simulink model "DYN_6DOF"  (R2018b)
(part 7 of 18)

+ 2*IPy6*the3_dot*cos(the2)*cos(the5)*sin(the3)*sin(the5)*sin(the6) + 2*IPy6*the3_dot*cos(the3)*cos(the5)*sin(the2)*sin(the5)*sin(the6) + IPy6*the5_dot*cos(the2)*cos(the6)*sin(the3)*sin(the4)*sin(the5) + IPy6*the5_dot*cos(the3)*cos(the6)*sin(the2)*sin(the4)*sin(the5) + IPy6*the6_dot*cos(the2)*cos(the5)*sin(the3)*sin(the4)*sin(the6) + IPy6*the6_dot*cos(the3)*cos(the5)*sin(the2)*sin(the4)*sin(the6) + 2*IPy6*the6_dot*cos(the5)*cos(the6)*sin(the2)*sin(the3)*sin(the5) + Ixx5*the2_dot*cos(the4)*cos(the5)*sin(the2)*sin(the3)*sin(the5) + Ixx5*the3_dot*cos(the4)*cos(the5)*sin(the2)*sin(the3)*sin(the5) + Ixx5*the4_dot*cos(the2)*cos(the5)*sin(the3)*sin(the4)*sin(the5) + Ixx5*the4_dot*cos(the3)*cos(the5)*sin(the2)*sin(the4)*sin(the5) - Iyy5*the2_dot*cos(the4)*cos(the5)*sin(the2)*sin(the3)*sin(the5) - Iyy5*the3_dot*cos(the4)*cos(the5)*sin(the2)*sin(the3)*sin(the5) + Iyy6*the2_dot*cos(the4)*cos(the5)*sin(the2)*sin(the3)*sin(the5) - Iyy5*the4_dot*cos(the2)*cos(the5)*sin(the3)*sin(the4)*sin(the5) - Iyy5*the4_dot*cos(the3)*cos(the5)*sin(the2)*sin(the4)*sin(the5) + Iyy6*the3_dot*cos(the4)*cos(the5)*sin(the2)*sin(the3)*sin(the5) + Iyy6*the4_dot*cos(the2)*cos(the5)*sin(the3)*sin(the4)*sin(the5) + Iyy6*the4_dot*cos(the3)*cos(the5)*sin(the2)*sin(the4)*sin(the5) - Izz6*the2_dot*cos(the4)*cos(the5)*sin(the2)*sin(the3)*sin(the5) - Izz6*the3_dot*cos(the4)*cos(the5)*sin(the2)*sin(the3)*sin(the5) - Izz6*the4_dot*cos(the2)*cos(the5)*sin(the3)*sin(the4)*sin(the5) - Izz6*the4_dot*cos(the3)*cos(the5)*sin(the2)*sin(the4)*sin(the5) + 2*m5*the5_dot*x5^2*cos(the2)*cos(the3)*cos(the5)*sin(the5) - 2*m6*the6_dot*x6^2*cos(the2)*cos(the3)*cos(the6)*sin(the6) - 2*m5*the5_dot*y5^2*cos(the2)*cos(the3)*cos(the5)*sin(the5) + 2*m6*the5_dot*y6^2*cos(the2)*cos(the3)*cos(the5)*sin(the5) + 2*m6*the6_dot*y6^2*cos(the2)*cos(the3)*cos(the6)*sin(the6) - 2*m6*the5_dot*z6^2*cos(the2)*cos(the3)*cos(the5)*sin(the5) + IPz6*the2_dot*cos(the5)*sin(the2)*sin(the3)*sin(the4)*sin(the6) + IPz6*the3_dot*cos(the5)*sin(the2)*sin(the3)*sin(the4)*sin(the6) + IPz6*the5_dot*cos(the2)*sin(the3)*sin(the4)*sin(the5)*sin(the6) + IPz6*the5_dot*cos(the3)*sin(the2)*sin(the4)*sin(the5)*sin(the6) + 2*IPz6*the6_dot*cos(the5)*sin(the2)*sin(the3)*sin(the5)*sin(the6) + a3*m4*the4_dot*y4*cos(the2)*cos(the3)*cos(the4) + a2*m5*the5_dot*y5*cos(the2)*cos(the4)*cos(the5) + a2*m6*the4_dot*y6*cos(the2)*cos(the4)*cos(the6) + a1*m6*the6_dot*y6*cos(the4)*cos(the5)*cos(the6) - a3*m5*the4_dot*z5*cos(the2)*cos(the3)*cos(the4) + a2*m6*the5_dot*z6*cos(the2)*cos(the4)*cos(the5) + d4*m4*the2_dot*x4*cos(the2)*cos(the3)*cos(the4) + d4*m4*the3_dot*x4*cos(the2)*cos(the3)*cos(the4) - 2*m5*the5_dot*x5^2*cos(the5)*sin(the2)*sin(the3)*sin(the5) + m6*the6_dot*x6^2*cos(the2)*sin(the3)*sin(the4)*sin(the5) + m6*the6_dot*x6^2*cos(the3)*sin(the2)*sin(the4)*sin(the5) + 2*m6*the6_dot*x6^2*cos(the6)*sin(the2)*sin(the3)*sin(the6) + 2*m5*the5_dot*y5^2*cos(the5)*sin(the2)*sin(the3)*sin(the5) - 2*m6*the5_dot*y6^2*cos(the5)*sin(the2)*sin(the3)*sin(the5) - m6*the6_dot*y6^2*cos(the2)*sin(the3)*sin(the4)*sin(the5) - m6*the6_dot*y6^2*cos(the3)*sin(the2)*sin(the4)*sin(the5) - 2*m6*the6_dot*y6^2*cos(the6)*sin(the2)*sin(the3)*sin(the6) + 2*m6*the5_dot*z6^2*cos(the5)*sin(the2)*sin(the3)*sin(the5) + a3*m4*the2_dot*x4*cos(the2)*cos(the4)*sin(the3) + a3*m4*the2_dot*x4*cos(the3)*cos(the4)*sin(the2) + a3*m4*the3_dot*x4*cos(the2)*cos(the4)*sin(the3) + a3*m4*the3_dot*x4*cos(the3)*cos(the4)*sin(the2) + a3*m4*the4_dot*x4*cos(the2)*cos(the3)*sin(the4) + a2*m5*the2_dot*x5*cos(the4)*cos(the5)*sin(the2) + a2*m5*the4_dot*x5*cos(the2)*cos(the5)*sin(the4) + a2*m5*the5_dot*x5*cos(the2)*cos(the4)*sin(the5) + a2*m6*the4_dot*x6*cos(the2)*cos(the4)*sin(the6) + a1*m6*the4_dot*x6*cos(the5)*cos(the6)*sin(the4) + a2*m6*the6_dot*x6*cos(the2)*cos(the6)*sin(the4) + a1*m6*the5_dot*x6*cos(the4)*cos(the6)*sin(the5) + a1*m6*the6_dot*x6*cos(the4)*cos(the5)*sin(the6) + 2*IPz6*the2_dot*cos(the2)*cos(the3)*cos(the4)*cos(the5)^2*cos(the6) + 2*IPz6*the3_dot*cos(the2)*cos(the3)*cos(the4)*cos(the5)^2*cos(the6) - d4*m4*the2_dot*y4*cos(the2)*cos(the3)*sin(the4) - d4*m4*the3_dot*y4*cos(the2)*cos(the3)*sin(the4) - d4*m4*the4_dot*y4*cos(the2)*cos(the4)*sin(the3) - d4*m4*the4_dot*y4*cos(the3)*cos(the4)*sin(the2) + d4*m5*the2_dot*z5*cos(the2)*cos(the3)*sin(the4) + d4*m5*the3_dot*z5*cos(the2)*cos(the3)*sin(the4) + d4*m5*the4_dot*z5*cos(the2)*cos(the4)*sin(the3) + d4*m5*the4_dot*z5*cos(the3)*cos(the4)*sin(the2) - m5*the2_dot*x5*y5*cos(the2)*cos(the3)*cos(the4) - m5*the3_dot*x5*y5*cos(the2)*cos(the3)*cos(the4) + m4*the2_dot*x4*z4*cos(the2)*cos(the3)*cos(the4) + m4*the3_dot*x4*z4*cos(the2)*cos(the3)*cos(the4) - 2*m6*the5_dot*x6*z6*cos(the2)*cos(the3)*cos(the6) - a3*m4*the2_dot*y4*cos(the2)*sin(the3)*sin(the4) - a3*m4*the2_dot*y4*cos(the3)*sin(the2)*sin(the4) - a3*m4*the3_dot*y4*cos(the2)*sin(the3)*sin(the4) - a3*m4*the3_dot*y4*cos(the3)*sin(the2)*sin(the4) - a3*m4*the4_dot*y4*cos(the4)*sin(the2)*sin(the3) - a2*m5*the2_dot*y5*cos(the4)*sin(the2)*sin(the5) - a2*m5*the4_dot*y5*cos(the2)*sin(the4)*sin(the5) - a2*m6*the2_dot*y6*cos(the6)*sin(the2)*sin(the4) - a1*m6*the4_dot*y6*cos(the5)*sin(the4)*sin(the6) - a2*m6*the6_dot*y6*cos(the2)*sin(the4)*sin(the6) - a1*m6*the5_dot*y6*cos(the4)*sin(the5)*sin(the6) + a3*m5*the2_dot*z5*cos(the2)*sin(the3)*sin(the4) + a3*m5*the2_dot*z5*cos(the3)*sin(the2)*sin(the4) + a3*m5*the3_dot*z5*cos(the2)*sin(the3)*sin(the4) + a3*m5*the3_dot*z5*cos(the3)*sin(the2)*sin(the4) + a3*m5*the4_dot*z5*cos(the4)*sin(the2)*sin(the3) - a2*m6*the2_dot*z6*cos(the4)*sin(the2)*sin(the5) - a2*m6*the4_dot*z6*cos(the2)*sin(the4)*sin(the5) - 2*IPy6*the2_dot*cos(the2)*cos(the3)*cos(the4)*cos(the5)^2*sin(the6) - 2*IPy6*the3_dot*cos(the2)*cos(the3)*cos(the4)*cos(the5)^2*sin(the6) - 2*IPy6*the6_dot*cos(the2)*cos(the4)*cos(the5)^2*cos(the6)*sin(the3) - 2*IPy6*the6_dot*cos(the3)*cos(the4)*cos(the5)^2*cos(the6)*sin(the2) - 2*Ixx6*the5_dot*cos(the2)*cos(the3)*cos(the5)*cos(the6)^2*sin(the5) - 2*Ixx6*the6_dot*cos(the2)*cos(the3)*cos(the5)^2*cos(the6)*sin(the6) + 2*Iyy6*the5_dot*cos(the2)*cos(the3)*cos(the5)*cos(the6)^2*sin(the5) + 2*Iyy6*the6_dot*cos(the2)*cos(the3)*cos(the5)^2*cos(the6)*sin(the6) - d4*m4*the2_dot*x4*cos(the4)*sin(the2)*sin(the3) - d4*m4*the3_dot*x4*cos(the4)*sin(the2)*sin(the3) - d4*m4*the4_dot*x4*cos(the2)*sin(the3)*sin(the4) - d4*m4*the4_dot*x4*cos(the3)*sin(the2)*sin(the4) - m4*the2_dot*y4*z4*cos(the2)*cos(the3)*sin(the4) - m4*the3_dot*y4*z4*cos(the2)*cos(the3)*sin(the4) - m4*the4_dot*y4*z4*cos(the2)*cos(the4)*sin(the3) - m4*the4_dot*y4*z4*cos(the3)*cos(the4)*sin(the2) + 2*m6*the5_dot*y6*z6*cos(the2)*cos(the3)*sin(the6) - a3*m4*the4_dot*x4*sin(the2)*sin(the3)*sin(the4) - a2*m6*the2_dot*x6*sin(the2)*sin(the4)*sin(the6) - 2*IPx6*the2_dot*cos(the2)*cos(the3)*cos(the6)^2*sin(the4)*sin(the5) - 2*IPx6*the3_dot*cos(the2)*cos(the3)*cos(the6)^2*sin(the4)*sin(the5) - 2*IPx6*the2_dot*cos(the2)*cos(the5)^2*cos(the6)*sin(the3)*sin(the6) - 2*IPx6*the2_dot*cos(the3)*cos(the5)^2*cos(the6)*sin(the2)*sin(the6) - 2*IPx6*the4_dot*cos(the2)*cos(the4)*cos(the6)^2*sin(the3)*sin(the5) - 2*IPx6*the4_dot*cos(the3)*cos(the4)*cos(the6)^2*sin(the2)*sin(the5) - 2*IPx6*the3_dot*cos(the2)*cos(the5)^2*cos(the6)*sin(the3)*sin(the6) - 2*IPx6*the3_dot*cos(the3)*cos(the5)^2*cos(the6)*sin(the2)*sin(the6) - 2*IPx6*the5_dot*cos(the2)*cos(the5)*cos(the6)^2*sin(the3)*sin(the4) - 2*IPx6*the5_dot*cos(the3)*cos(the5)*cos(the6)^2*sin(the2)*sin(the4) - 2*IPz6*the2_dot*cos(the4)*cos(the5)^2*cos(the6)*sin(the2)*sin(the3) - 2*IPz6*the3_dot*cos(the4)*cos(the5)^2*cos(the6)*sin(the2)*sin(the3) - 2*IPz6*the4_dot*cos(the2)*cos(the5)^2*cos(the6)*sin(the3)*sin(the4) - 2*IPz6*the4_dot*cos(the3)*cos(the5)^2*cos(the6)*sin(the2)*sin(the4) - 2*IPz6*the6_dot*cos(the2)*cos(the4)*cos(the5)^2*sin(the3)*sin(the6) - 2*IPz6*the6_dot*cos(the3)*cos(the4)*cos(the5)^2*sin(the2)*sin(the6) + d4*m4*the2_dot*y4*sin(the2)*sin(the3)*sin(the4) + d4*m4*the3_dot*y4*sin(the2)*sin(the3)*sin(the4) - d4*m5*the2_dot*z5*sin(the2)*sin(the3)*sin(the4) - d4*m5*the3_dot*z5*sin(the2)*sin(the3)*sin(the4) + m5*the2_dot*x5*y5*cos(the4)*sin(the2)*sin(the3) + m5*the3_dot*x5*y5*cos(the4)*sin(the2)*sin(the3) + m5*the4_dot*x5*y5*cos(the2)*sin(the3)*sin(the4) + m5*the4_dot*x5*y5*cos(the3)*sin(the2)*sin(the4) - m4*the2_dot*x4*z4*cos(the4)*sin(the2)*sin(the3) - m4*the3_dot*x4*z4*cos(the4)*sin(the2)*sin(the3) - m4*the4_dot*x4*z4*cos(the2)*sin(the3)*sin(the4) - m4*the4_dot*x4*z4*cos(the3)*sin(the2)*sin(the4) + 2*m6*the5_dot*x6*z6*cos(the6)*sin(the2)*sin(the3) + 2*IPy6*the2_dot*cos(the4)*cos(the5)^2*sin(the2)*sin(the3)*sin(the6) + 2*IPy6*the3_dot*cos(the4)*cos(the5)^2*sin(the2)*sin(the3)*sin(the6) + 2*IPy6*the4_dot*cos(the2)*cos(the5)^2*sin(the3)*sin(the4)*sin(the6) + 2*IPy6*the4_dot*cos(the3)*cos(the5)^2*sin(the2)*sin(the4)*sin(the6) + 2*Ixx6*the5_dot*cos(the5)*cos(the6)^2*sin(the2)*sin(the3)*sin(the5) + 2*Ixx6*the6_dot*cos(the2)*cos(the6)^2*sin(the3)*sin(the4)*sin(the5) + 2*Ixx6*the6_dot*cos(the3)*cos(the6)^2*sin(the2)*sin(the4)*sin(the5) + 2*Ixx6*the6_dot*cos(the5)^2*cos(the6)*sin(the2)*sin(the3)*sin(the6) - 2*Iyy6*the5_dot*cos(the5)*cos(the6)^2*sin(the2)*sin(the3)*sin(the5) - 2*Iyy6*the6_dot*cos(the2)*cos(the6)^2*sin(the3)*sin(the4)*sin(the5) - 2*Iyy6*the6_dot*cos(the3)*cos(the6)^2*sin(the2)*sin(the4)*sin(the5) - 2*Iyy6*the6_dot*cos(the5)^2*cos(the6)*sin(the2)*sin(the3)*sin(the6) + 2*m5*the5_dot*x5^2*cos(the2)*cos(the4)*cos(the5)^2*sin(the3) + 2*m5*the5_dot*x5^2*cos(the3)*cos(the4)*cos(the5)^2*sin(the2) - m6*the5_dot*x6^2*cos(the2)*cos(the4)*cos(the6)^2*sin(the3) - m6*the5_dot*x6^2*cos(the3)*cos(the4)*cos(the6)^2*sin(the2) - 2*m5*the5_dot*y5^2*cos(the2)*cos(the4)*cos(the5)^2*sin(the3) - 2*m5*the5_dot*y5^2*cos(the3)*cos(the4)*cos(the5)^2*sin(the2) + 2*m6*the5_dot*y6^2*cos(the2)*cos(the4)*cos(the5)^2*sin(the3) + 2*m6*the5_dot*y6^2*cos(the3)*cos(the4)*cos(the5)^2*sin(the2) + m6*the5_dot*y6^2*cos(the2)*cos(the4)*cos(the6)^2*sin(the3) + m6*the5_dot*y6^2*cos(the3)*cos(the4)*cos(the6)^2*sin(the2) - 2*m6*the5_dot*z6^2*cos(the2)*cos(the4)*cos(the5)^2*sin(the3) - 2*m6*the5_dot*z6^2*cos(the3)*cos(the4)*cos(the5)^2*sin(the2) + m4*the2_dot*y4*z4*sin(the2)*sin(the3)*sin(the4) + m4*the3_dot*y4*z4*sin(the2)*sin(the3)*sin(the4) - 2*m6*the5_dot*y6*z6*sin(the2)*sin(the3)*sin(the6) + 2*IPx6*the2_dot*cos(the6)^2*sin(the2)*sin(the3)*sin(the4)*sin(the5) + 2*IPx6*the3_dot*cos(the6)^2*sin(the2)*sin(the3)*sin(the4)*sin(the5) - 4*m6*the5_dot*y6*z6*cos(the2)*cos(the3)*cos(the5)^2*sin(the6) - 2*m5*the2_dot*x5*y5*cos(the4)*cos(the5)^2*sin(the2)*sin(the3) - 2*m5*the3_dot*x5*y5*cos(the4)*cos(the5)^2*sin(the2)*sin(the3) - 2*m5*the4_dot*x5*y5*cos(the2)*cos(the5)^2*sin(the3)*sin(the4) - 2*m5*the4_dot*x5*y5*cos(the3)*cos(the5)^2*sin(the2)*sin(the4) - 4*m6*the5_dot*x6*z6*cos(the5)^2*cos(the6)*sin(the2)*sin(the3) + 2*m6*the5_dot*x6^2*cos(the2)*cos(the4)*cos(the5)^2*cos(the6)^2*sin(the3) + 2*m6*the5_dot*x6^2*cos(the3)*cos(the4)*cos(the5)^2*cos(the6)^2*sin(the2) - 2*m6*the5_dot*y6^2*cos(the2)*cos(the4)*cos(the5)^2*cos(the6)^2*sin(the3) - 2*m6*the5_dot*y6^2*cos(the3)*cos(the4)*cos(the5)^2*cos(the6)^2*sin(the2) + 4*m6*the5_dot*y6*z6*cos(the5)^2*sin(the2)*sin(the3)*sin(the6) - 4*IPx6*the5_dot*cos(the2)*cos(the3)*cos(the5)*cos(the6)*sin(the5)*sin(the6) - 4*IPz6*the5_dot*cos(the2)*cos(the4)*cos(the5)*cos(the6)*sin(the3)*sin(the5) - 4*IPz6*the5_dot*cos(the3)*cos(the4)*cos(the5)*cos(the6)*sin(the2)*sin(the5) + 4*m6*the6_dot*x6*y6*cos(the2)*cos(the3)*cos(the5)^2*cos(the6)^2 + 4*IPy6*the5_dot*cos(the2)*cos(the4)*cos(the5)*sin(the3)*sin(the5)*sin(the6) + 4*IPy6*the5_dot*cos(the3)*cos(the4)*cos(the5)*sin(the2)*sin(the5)*sin(the6) + Ixx6*the2_dot*cos(the2)*cos(the3)*cos(the6)*sin(the4)*sin(the5)*sin(the6) + Ixx6*the3_dot*cos(the2)*cos(the3)*cos(the6)*sin(the4)*sin(the5)*sin(the6) + Ixx6*the4_dot*cos(the2)*cos(the4)*cos(the6)*sin(the3)*sin(the5)*sin(the6) + Ixx6*the4_dot*cos(the3)*cos(the4)*cos(the6)*sin(the2)*sin(the5)*sin(the6) + Ixx6*the5_dot*cos(the2)*cos(the5)*cos(the6)*sin(the3)*sin(the4)*sin(the6) + Ixx6*the5_dot*cos(the3)*cos(the5)*cos(the6)*sin(the2)*sin(the4)*sin(the6) - Iyy6*the2_dot*cos(the2)*cos(the3)*cos(the6)*sin(the4)*sin(the5)*sin(the6) - Iyy6*the3_dot*cos(the2)*cos(the3)*cos(the6)*sin(the4)*sin(the5)*sin(the6) - Iyy6*the4_dot*cos(the2)*cos(the4)*cos(the6)*sin(the3)*sin(the5)*sin(the6) - Iyy6*the4_dot*cos(the3)*cos(the4)*cos(the6)*sin(the2)*sin(the5)*sin(the6) - Iyy6*the5_dot*cos(the2)*cos(the5)*cos(the6)*sin(the3)*sin(the4)*sin(the6) - Iyy6*the5_dot*cos(the3)*cos(the5)*cos(the6)*sin(the2)*sin(the4)*sin(the6) + m5*the2_dot*x5^2*cos(the2)*cos(the3)*cos(the4)*cos(the5)*sin(the5) + m5*the3_dot*x5^2*cos(the2)*cos(the3)*cos(the4)*cos(the5)*sin(the5) - m5*the2_dot*y5^2*cos(the2)*cos(the3)*cos(the4)*cos(the5)*sin(the5) - m5*the3_dot*y5^2*cos(the2)*cos(the3)*cos(the4)*cos(the5)*sin(the5) + m6*the2_dot*y6^2*cos(the2)*cos(the3)*cos(the4)*cos(the5)*sin(the5) + m6*the3_dot*y6^2*cos(the2)*cos(the3)*cos(the4)*cos(the5)*sin(the5) - m6*the2_dot*z6^2*cos(the2)*cos(the3)*cos(the4)*cos(the5)*sin(the5) - m6*the3_dot*z6^2*cos(the2)*cos(the3)*cos(the4)*cos(the5)*sin(the5) + 4*IPx6*the5_dot*cos(the5)*cos(the6)*sin(the2)*sin(the3)*sin(the5)*sin(the6) + 4*IPx6*the6_dot*cos(the2)*cos(the6)*sin(the3)*sin(the4)*sin(the5)*sin(the6) + 4*IPx6*the6_dot*cos(the3)*cos(the6)*sin(the2)*sin(the4)*sin(the5)*sin(the6) - 4*m6*the6_dot*x6*y6*cos(the5)^2*cos(the6)^2*sin(the2)*sin(the3) + a3*m5*the5_dot*y5*cos(the2)*cos(the3)*cos(the4)*cos(the5) + a3*m6*the4_dot*y6*cos(the2)*cos(the3)*cos(the4)*cos(the6) + a2*m6*the6_dot*y6*cos(the2)*cos(the4)*cos(the5)*cos(the6) + a3*m6*the5_dot*z6*cos(the2)*cos(the3)*cos(the4)*cos(the5) + d4*m5*the2_dot*x5*cos(the2)*cos(the3)*cos(the4)*cos(the5) + d4*m5*the3_dot*x5*cos(the2)*cos(the3)*cos(the4)*cos(the5) - Ixx6*the2_dot*cos(the6)*sin(the2)*sin(the3)*sin(the4)*sin(the5)*sin(the6) - Ixx6*the3_dot*cos(the6)*sin(the2)*sin(the3)*sin(the4)*sin(the5)*sin(the6) + Iyy6*the2_dot*cos(the6)*sin(the2)*sin(the3)*sin(the4)*sin(the5)*sin(the6) + Iyy6*the3_dot*cos(the6)*sin(the2)*sin(the3)*sin(the4)*sin(the5)*sin(the6) - m5*the2_dot*x5^2*cos(the4)*cos(the5)*sin(the2)*sin(the3)*sin(the5) - m5*the3_dot*x5^2*cos(the4)*cos(the5)*sin(the2)*sin(the3)*sin(the5) - m5*the4_dot*x5^2*cos(the2)*cos(the5)*sin(the3)*sin(the4)*sin(the5) - m5*the4_dot*x5^2*cos(the3)*cos(the5)*sin(the2)*sin(the4)*sin(the5) + m5*the2_dot*y5^2*cos(the4)*cos(the5)*sin(the2)*sin(the3)*sin(the5) + m5*the3_dot*y5^2*cos(the4)*cos(the5)*sin(the2)*sin(the3)*sin(the5) + m5*the4_dot*y5^2*cos(the2)*cos(the5)*sin(the3)*sin(the4)*sin(the5) + m5*the4_dot*y5^2*cos(the3)*cos(the5)*sin(the2)*sin(the4)*sin(the5) - m6*the2_dot*y6^2*cos(the4)*cos(the5)*sin(the2)*sin(the3)*sin(the5) - m6*the3_dot*y6^2*cos(the4)*cos(the5)*sin(the2)*sin(the3)*sin(the5) - m6*the4_dot*y6^2*cos(the2)*cos(the5)*sin(the3)*sin(the4)*sin(the5) - m6*the4_dot*y6^2*cos(the3)*cos(the5)*sin(the2)*sin(the4)*sin(the5) + m6*the2_dot*z6^2*cos(the4)*cos(the5)*sin(the2)*sin(the3)*sin(the5) + m6*the3_dot*z6^2*cos(the4)*cos(the5)*sin(the2)*sin(the3)*sin(the5) + m6*the4_dot*z6^2*cos(the2)*cos(the5)*sin(the3)*sin(the4)*sin(the5) + m6*the4_dot*z6^2*cos(the3)*cos(the5)*sin(the2)*sin(the4)*sin(the5) + a3*m5*the2_dot*x5*cos(the2)*cos(the4)*cos(the5)*sin(the3) + a3*m5*the2_dot*x5*cos(the3)*cos(the4)*cos(the5)*sin(the2) + a3*m5*the3_dot*x5*cos(the2)*cos(the4)*cos(the5)*sin(the3) + a3*m5*the3_dot*x5*cos(the3)*cos(the4)*cos(the5)*sin(the2) + a3*m5*the4_dot*x5*cos(the2)*cos(the3)*cos(the5)*sin(the4) + a3*m5*the5_dot*x5*cos(the2)*cos(the3)*cos(the4)*sin(the5) + a2*m6*the2_dot*x6*cos(the4)*cos(the5)*cos(the6)*sin(the2) + a3*m6*the4_dot*x6*cos(the2)*cos(the3)*cos(the4)*sin(the6) + a2*m6*the4_dot*x6*cos(the2)*cos(the5)*cos(the6)*sin(the4) + a2*m6*the5_dot*x6*cos(the2)*cos(the4)*cos(the6)*sin(the5) + a3*m6*the6_dot*x6*cos(the2)*cos(the3)*cos(the6)*sin(the4) + a2*m6*the6_dot*x6*cos(the2)*cos(the4)*cos(the5)*sin(the6) - d4*m5*the2_dot*y5*cos(the2)*cos(the3)*cos(the4)*sin(the5) - d4*m5*the3_dot*y5*cos(the2)*cos(the3)*cos(the4)*sin(the5) - d4*m5*the5_dot*y5*cos(the2)*cos(the4)*cos(the5)*sin(the3) - d4*m5*the5_dot*y5*cos(the3)*cos(the4)*cos(the5)*sin(the2) - d4*m6*the2_dot*y6*cos(the2)*cos(the3)*cos(the6)*sin(the4) - d4*m6*the3_dot*y6*cos(the2)*cos(the3)*cos(the6)*sin(the4) - d4*m6*the4_dot*y6*cos(the2)*cos(the4)*cos(the6)*sin(the3) - d4*m6*the4_dot*y6*cos(the3)*cos(the4)*cos(the6)*sin(the2) - d4*m6*the2_dot*z6*cos(the2)*cos(the3)*cos(the4)*sin(the5) - d4*m6*the3_dot*z6*cos(the2)*cos(the3)*cos(the4)*sin(the5) - d4*m6*the5_dot*z6*cos(the2)*cos(the4)*cos(the5)*sin(the3) - d4*m6*the5_dot*z6*cos(the3)*cos(the4)*cos(the5)*sin(the2) - m6*the2_dot*x6*z6*cos(the2)*cos(the3)*cos(the4)*cos(the6) - m6*the3_dot*x6*z6*cos(the2)*cos(the3)*cos(the4)*cos(the6) - a3*m5*the2_dot*y5*cos(the2)*cos(the4)*sin(the3)*sin(the5) - a3*m5*the2_dot*y5*cos(the3)*cos(the4)*sin(the2)*sin(the5) - a3*m5*the3_dot*y5*cos(the2)*cos(the4)*sin(the3)*sin(the5) - a3*m5*the3_dot*y5*cos(the3)*cos(the4)*sin(the2)*sin(the5) - a3*m5*the4_dot*y5*cos(the2)*cos(the3)*sin(the4)*sin(the5) - a3*m5*the5_dot*y5*cos(the4)*cos(the5)*sin(the2)*sin(the3) - a3*m6*the2_dot*y6*cos(the2)*cos(the6)*sin(the3)*sin(the4) - a3*m6*the2_dot*y6*cos(the3)*cos(the6)*sin(the2)*sin(the4) - a2*m6*the2_dot*y6*cos(the4)*cos(the5)*sin(the2)*sin(the6) - a3*m6*the3_dot*y6*cos(the2)*cos(the6)*sin(the3)*sin(the4) - a3*m6*the3_dot*y6*cos(the3)*cos(the6)*sin(the2)*sin(the4) - a3*m6*the4_dot*y6*cos(the4)*cos(the6)*sin(the2)*sin(the3) - a2*m6*the4_dot*y6*cos(the2)*cos(the5)*sin(the4)*sin(the6) - a2*m6*the5_dot*y6*cos(the2)*cos(the4)*sin(the5)*sin(the6) - a3*m6*the6_dot*y6*cos(the2)*cos(the3)*sin(the4)*sin(the6) - a3*m6*the2_dot*z6*cos(the2)*cos(the4)*sin(the3)*sin(the5) - a3*m6*the2_dot*z6*cos(the3)*cos(the4)*sin(the2)*sin(the5) - a3*m6*the3_dot*z6*cos(the2)*cos(the4)*sin(the3)*sin(the5) - a3*m6*the3_dot*z6*cos(the3)*cos(the4)*sin(the2)*sin(the5) - a3*m6*the4_dot*z6*cos(the2)*cos(the3)*sin(the4)*sin(the5) - a3*m6*the5_dot*z6*cos(the4)*cos(the5)*sin(the2)*sin(the3) - Ixx6*the2_dot*cos(the2)*cos(the3)*cos(the4)*cos(the5)*cos(the6)^2*sin(the5) - Ixx6*the3_dot*cos(the2)*cos(the3)*cos(the4)*cos(the5)*cos(the6)^2*sin(the5) + Iyy6*the2_dot*cos(the2)*cos(the3)*cos(the4)*cos(the5)*cos(the6)^2*sin(the5) + Iyy6*the3_dot*cos(the2)*cos(the3)*cos(the4)*cos(the5)*cos(the6)^2*sin(the5) - d4*m5*the2_dot*x5*cos(the4)*cos(the5)*sin(the2)*sin(the3) - d4*m5*the3_dot*x5*cos(the4)*cos(the5)*sin(the2)*sin(the3) - d4*m5*the4_dot*x5*cos(the2)*cos(the5)*sin(the3)*sin(the4) - d4*m5*the4_dot*x5*cos(the3)*cos(the5)*sin(the2)*sin(the4) - d4*m5*the5_dot*x5*cos(the2)*cos(the4)*sin(the3)*sin(the5) - d4*m5*the5_dot*x5*cos(the3)*cos(the4)*sin(the2)*sin(the5) - d4*m6*the2_dot*x6*cos(the2)*cos(the3)*sin(the4)*sin(the6) - d4*m6*the3_dot*x6*cos(the2)*cos(the3)*sin(the4)*sin(the6) - d4*m6*the4_dot*x6*cos(the2)*cos(the4)*sin(the3)*sin(the6) - d4*m6*the4_dot*x6*cos(the3)*cos(the4)*sin(the2)*sin(the6) - d4*m6*the6_dot*x6*cos(the2)*cos(the6)*sin(the3)*sin(the4) - d4*m6*the6_dot*x6*cos(the3)*cos(the6)*sin(the2)*sin(the4) + m5*the2_dot*y5*z5*cos(the2)*cos(the3)*cos(the5)*sin(the4) + m5*the3_dot*y5*z5*cos(the2)*cos(the3)*cos(the5)*sin(the4) + m5*the4_dot*y5*z5*cos(the2)*cos(the4)*cos(the5)*sin(the3) + m5*the4_dot*y5*z5*cos(the3)*cos(the4)*cos(the5)*sin(the2) + m6*the2_dot*y6*z6*cos(the2)*cos(the3)*cos(the4)*sin(the6) + m6*the3_dot*y6*z6*cos(the2)*cos(the3)*cos(the4)*sin(the6) + m6*the6_dot*y6*z6*cos(the2)*cos(the4)*cos(the6)*sin(the3) + m6*the6_dot*y6*z6*cos(the3)*cos(the4)*cos(the6)*sin(the2) - a3*m5*the4_dot*x5*cos(the5)*sin(the2)*sin(the3)*sin(the4) - a3*m5*the5_dot*x5*cos(the4)*sin(the2)*sin(the3)*sin(the5) - a3*m6*the2_dot*x6*cos(the2)*sin(the3)*sin(the4)*sin(the6) - a3*m6*the2_dot*x6*cos(the3)*sin(the2)*sin(the4)*sin(the6) - a3*m6*the3_dot*x6*cos(the2)*sin(the3)*sin(the4)*sin(the6) - a3*m6*the3_dot*x6*cos(the3)*sin(the2)*sin(the4)*sin(the6) - a3*m6*the4_dot*x6*cos(the4)*sin(the2)*sin(the3)*sin(the6) - a3*m6*the6_dot*x6*cos(the6)*sin(the2)*sin(the3)*sin(the4) - 4*IPx6*the5_dot*cos(the2)*cos(the4)*cos(the5)^2*cos(the6)*sin(the3)*sin(the6) - 4*IPx6*the5_dot*cos(the3)*cos(the4)*cos(the5)^2*cos(the6)*sin(the2)*sin(the6) - 4*IPx6*the6_dot*cos(the2)*cos(the4)*cos(the5)*cos(the6)^2*sin(the3)*sin(the5) - 4*IPx6*the6_dot*cos(the3)*cos(the4)*cos(the5)*cos(the6)^2*sin(the2)*sin(the5) + d4*m5*the2_dot*y5*cos(the4)*sin(the2)*sin(the3)*sin(the5) + d4*m5*the3_dot*y5*cos(the4)*sin(the2)*sin(the3)*sin(the5) + d4*m5*the4_dot*y5*cos(the2)*sin(the3)*sin(the4)*sin(the5) + d4*m5*the4_dot*y5*cos(the3)*sin(the2)*sin(the4)*sin(the5) + d4*m6*the2_dot*y6*cos(the6)*sin(the2)*sin(the3)*sin(the4) + d4*m6*the3_dot*y6*cos(the6)*sin(the2)*sin(the3)*sin(the4) + d4*m6*the6_dot*y6*cos(the2)*sin(the3)*sin(the4)*sin(the6) + d4*m6*the6_dot*y6*cos(the3)*sin(the2)*sin(the4)*sin(the6) + d4*m6*the2_dot*z6*cos(the4)*sin(the2)*sin(the3)*sin(the5) + d4*m6*the3_dot*z6*cos(the4)*sin(the2)*sin(the3)*sin(the5) + d4*m6*the4_dot*z6*cos(the2)*sin(the3)*sin(the4)*sin(the5) + d4*m6*the4_dot*z6*cos(the3)*sin(the2)*sin(the4)*sin(the5) - 2*m5*the2_dot*x5*y5*cos(the2)*cos(the5)*sin(the3)*sin(the5) - 2*m5*the2_dot*x5*y5*cos(the3)*cos(the5)*sin(the2)*sin(the5) - 2*m5*the3_dot*x5*y5*cos(the2)*cos(the5)*sin(the3)*sin(the5) - 2*m5*the3_dot*x5*y5*cos(the3)*cos(the5)*sin(the2)*sin(the5) + m6*the2_dot*x6*y6*cos(the2)*cos(the3)*sin(the4)*sin(the5) + m6*the3_dot*x6*y6*cos(the2)*cos(the3)*sin(the4)*sin(the5) + m6*the4_dot*x6*y6*cos(the2)*cos(the4)*sin(the3)*sin(the5) + m6*the4_dot*x6*y6*cos(the3)*cos(the4)*sin(the2)*sin(the5) + 2*m6*the2_dot*x6*y6*cos(the2)*cos(the6)*sin(the3)*sin(the6) + 2*m6*the2_dot*x6*y6*cos(the3)*cos(the6)*sin(the2)*sin(the6) + m6*the5_dot*x6*y6*cos(the2)*cos(the5)*sin(the3)*sin(the4) + m6*the5_dot*x6*y6*cos(the3)*cos(the5)*sin(the2)*sin(the4) + 2*m6*the3_dot*x6*y6*cos(the2)*cos(the6)*sin(the3)*sin(the6) + 2*m6*the3_dot*x6*y6*cos(the3)*cos(the6)*sin(the2)*sin(the6) + m5*the2_dot*x5*z5*cos(the2)*cos(the3)*sin(the4)*sin(the5) + m5*the3_dot*x5*z5*cos(the2)*cos(the3)*sin(the4)*sin(the5) + m5*the4_dot*x5*z5*cos(the2)*cos(the4)*sin(the3)*sin(the5) + m5*the4_dot*x5*z5*cos(the3)*cos(the4)*sin(the2)*sin(the5) + m5*the5_dot*x5*z5*cos(the2)*cos(the5)*sin(the3)*sin(the4) + m5*the5_dot*x5*z5*cos(the3)*cos(the5)*sin(the2)*sin(the4) + m6*the2_dot*x6*z6*cos(the4)*cos(the6)*sin(the2)*sin(the3) + m6*the3_dot*x6*z6*cos(the4)*cos(the6)*sin(the2)*sin(the3) + m6*the4_dot*x6*z6*cos(the2)*cos(the6)*sin(the3)*sin(the4) + m6*the4_dot*x6*z6*cos(the3)*cos(the6)*sin(the2)*sin(the4) + m6*the6_dot*x6*z6*cos(the2)*cos(the4)*sin(the3)*sin(the6) + m6*the6_dot*x6*z6*cos(the3)*cos(the4)*sin(the2)*sin(the6) + a3*m5*the4_dot*y5*sin(the2)*sin(the3)*sin(the4)*sin(the5) + a3*m6*the6_dot*y6*sin(the2)*sin(the3)*sin(the4)*sin(the6) + a3*m6*the4_dot*z6*sin(the2)*sin(the3)*sin(the4)*sin(the5) + Ixx6*the2_dot*cos(the4)*cos(the5)*cos(the6)^2*sin(the2)*sin(the3)*sin(the5) + Ixx6*the3_dot*cos(the4)*cos(the5)*cos(the6)^2*sin(the2)*sin(the3)*sin(the5) + Ixx6*the4_dot*cos(the2)*cos(the5)*cos(the6)^2*sin(the3)*sin(the4)*sin(the5) + Ixx6*the4_dot*cos(the3)*cos(the5)*cos(the6)^2*sin(the2)*sin(the4)*sin(the5) - Iyy6*the2_dot*cos(the4)*cos(the5)*cos(the6)^2*sin(the2)*sin(the3)*sin(the5) - Iyy6*the3_dot*cos(the4)*cos(the5)*cos(the6)^2*sin(the2)*sin(the3)*sin(the5) - Iyy6*the4_dot*cos(the2)*cos(the5)*cos(the6)^2*sin(the3)*sin(the4)*sin(the5) - Iyy6*the4_dot*cos(the3)*cos(the5)*cos(the6)^2*sin(the2)*sin(the4)*sin(the5) + d4*m6*the2_dot*x6*sin(the2)*sin(the3)*sin(the4)*sin(the6) + d4*m6*the3_dot*x6*sin(the2)*sin(the3)*sin(the4)*sin(the6) + 2*m6*the5_dot*x6^2*cos(the2)*cos(the3)*cos(the5)*cos(the6)^2*sin(the5) + 2*m6*the6_dot*x6^2*cos(the2)*cos(the3)*cos(the5)^2*cos(the6)*sin(the6) - 2*m6*the5_dot*y6^2*cos(the2)*cos(the3)*cos(the5)*cos(the6)^2*sin(the5) - 2*m6*the6_dot*y6^2*cos(the2)*cos(the3)*cos(the5)^2*cos(the6)*sin(the6) - m5*the2_dot*y5*z5*cos(the5)*sin(the2)*sin(the3)*sin(the4) - m5*the3_dot*y5*z5*cos(the5)*sin(the2)*sin(the3)*sin(the4) - m5*the5_dot*y5*z5*cos(the2)*sin(the3)*sin(the4)*sin(the5) - m5*the5_dot*y5*z5*cos(the3)*sin(the2)*sin(the4)*sin(the5) - m6*the2_dot*y6*z6*cos(the4)*sin(the2)*sin(the3)*sin(the6) - m6*the3_dot*y6*z6*cos(the4)*sin(the2)*sin(the3)*sin(the6) - m6*the4_dot*y6*z6*cos(the2)*sin(the3)*sin(the4)*sin(the6) - m6*the4_dot*y6*z6*cos(the3)*sin(the2)*sin(the4)*sin(the6) - m6*the2_dot*x6*y6*sin(the2)*sin(the3)*sin(the4)*sin(the5) - m6*the3_dot*x6*y6*sin(the2)*sin(the3)*sin(the4)*sin(the5) - m5*the2_dot*x5*z5*sin(the2)*sin(the3)*sin(the4)*sin(the5) - m5*the3_dot*x5*z5*sin(the2)*sin(the3)*sin(the4)*sin(the5) - 2*m6*the5_dot*x6^2*cos(the5)*cos(the6)^2*sin(the2)*sin(the3)*sin(the5) - 2*m6*the6_dot*x6^2*cos(the2)*cos(the6)^2*sin(the3)*sin(the4)*sin(the5) - 2*m6*the6_dot*x6^2*cos(the3)*cos(the6)^2*sin(the2)*sin(the4)*sin(the5) - 2*m6*the6_dot*x6^2*cos(the5)^2*cos(the6)*sin(the2)*sin(the3)*sin(the6) + 2*m6*the5_dot*y6^2*cos(the5)*cos(the6)^2*sin(the2)*sin(the3)*sin(the5) + 2*m6*the6_dot*y6^2*cos(the2)*cos(the6)^2*sin(the3)*sin(the4)*sin(the5) + 2*m6*the6_dot*y6^2*cos(the3)*cos(the6)^2*sin(the2)*sin(the4)*sin(the5) + 2*m6*the6_dot*y6^2*cos(the5)^2*cos(the6)*sin(the2)*sin(the3)*sin(the6) + 2*m5*the2_dot*x5*y5*cos(the2)*cos(the3)*cos(the4)*cos(the5)^2 + 2*m5*the3_dot*x5*y5*cos(the2)*cos(the3)*cos(the4)*cos(the5)^2 + 4*m6*the5_dot*x6*z6*cos(the2)*cos(the3)*cos(the5)^2*cos(the6) + 2*m6*the2_dot*x6*y6*cos(the6)^2*sin(the2)*sin(the3)*sin(the4)*sin(the5) + 2*m6*the3_dot*x6*y6*cos(the6)^2*sin(the2)*sin(the3)*sin(the4)*sin(the5) - 2*IPx6*the2_dot*cos(the2)*cos(the3)*cos(the4)*cos(the5)*cos(the6)*sin(the5)*sin(the6) - 2*IPx6*the3_dot*cos(the2)*cos(the3)*cos(the4)*cos(the5)*cos(the6)*sin(the5)*sin(the6) + 2*Ixx6*the6_dot*cos(the2)*cos(the4)*cos(the5)*cos(the6)*sin(the3)*sin(the5)*sin(the6) + 2*Ixx6*the6_dot*cos(the3)*cos(the4)*cos(the5)*cos(the6)*sin(the2)*sin(the5)*sin(the6) - 2*Iyy6*the6_dot*cos(the2)*cos(the4)*cos(the5)*cos(the6)*sin(the3)*sin(the5)*sin(the6) - 2*Iyy6*the6_dot*cos(the3)*cos(the4)*cos(the5)*cos(the6)*sin(the2)*sin(the5)*sin(the6) + 2*IPx6*the2_dot*cos(the4)*cos(the5)*cos(the6)*sin(the2)*sin(the3)*sin(the5)*sin(the6) + 2*IPx6*the3_dot*cos(the4)*cos(the5)*cos(the6)*sin(the2)*sin(the3)*sin(the5)*sin(the6) + 2*IPx6*the4_dot*cos(the2)*cos(the5)*cos(the6)*sin(the3)*sin(the4)*sin(the5)*sin(the6) + 2*IPx6*the4_dot*cos(the3)*cos(the5)*cos(the6)*sin(the2)*sin(the4)*sin(the5)*sin(the6) + a3*m6*the6_dot*y6*cos(the2)*cos(the3)*cos(the4)*cos(the5)*cos(the6) + d4*m6*the2_dot*x6*cos(the2)*cos(the3)*cos(the4)*cos(the5)*cos(the6) + d4*m6*the3_dot*x6*cos(the2)*cos(the3)*cos(the4)*cos(the5)*cos(the6) - m6*the2_dot*x6^2*cos(the2)*cos(the3)*cos(the6)*sin(the4)*sin(the5)*sin(the6) - m6*the3_dot*x6^2*cos(the2)*cos(the3)*cos(the6)*sin(the4)*sin(the5)*sin(the6) - m6*the4_dot*x6^2*cos(the2)*cos(the4)*cos(the6)*sin(the3)*sin(the5)*sin(the6) - m6*the4_dot*x6^2*cos(the3)*cos(the4)*cos(the6)*sin(the2)*sin(the5)*sin(the6) - m6*the5_dot*x6^2*cos(the2)*cos(the5)*cos(the6)*sin(the3)*sin(the4)*sin(the6) - m6*the5_dot*x6^2*cos(the3)*cos(the5)*cos(the6)*sin(the2)*sin(the4)*sin(the6) + m6*the2_dot*y6^2*cos(the2)*cos(the3)*cos(the6)*sin(the4)*sin(the5)*sin(the6) + m6*the3_dot*y6^2*cos(the2)*cos(the3)*cos(the6)*sin(the4)*sin(the5)*sin(the6) + m6*the4_dot*y6^2*cos(the2)*cos(the4)*cos(the6)*sin(the3)*sin(the5)*sin(the6) + m6*the4_dot*y6^2*cos(the3)*cos(the4)*cos(the6)*sin(the2)*sin(the5)*sin(the6) + m6*the5_dot*y6^2*cos(the2)*cos(the5)*cos(the6)*sin(the3)*sin(the4)*sin(the6) + m6*the5_dot*y6^2*cos(the3)*cos(the5)*cos(the6)*sin(the2)*sin(the4)*sin(the6) + a3*m6*the2_dot*x6*cos(the2)*cos(the4)*cos(the5)*cos(the6)*sin(the3) + a3*m6*the2_dot*x6*cos(the3)*cos(the4)*cos(the5)*cos(the6)*sin(the2) + a3*m6*the3_dot*x6*cos(the2)*cos(the4)*cos(the5)*cos(the6)*sin(the3) + a3*m6*the3_dot*x6*cos(the3)*cos(the4)*cos(the5)*cos(the6)*sin(the2) + a3*m6*the4_dot*x6*cos(the2)*cos(the3)*cos(the5)*cos(the6)*sin(the4) + a3*m6*the5_dot*x6*cos(the2)*cos(the3)*cos(the4)*cos(the6)*sin(the5) + a3*m6*the6_dot*x6*cos(the2)*cos(the3)*cos(the4)*cos(the5)*sin(the6) - d4*m6*the2_dot*y6*cos(the2)*cos(the3)*cos(the4)*cos(the5)*sin(the6) - d4*m6*the3_dot*y6*cos(the2)*cos(the3)*cos(the4)*cos(the5)*sin(the6) - d4*m6*the6_dot*y6*cos(the2)*cos(the4)*cos(the5)*cos(the6)*sin(the3) - d4*m6*the6_dot*y6*cos(the3)*cos(the4)*cos(the5)*cos(the6)*sin(the2) - a3*m6*the2_dot*y6*cos(the2)*cos(the4)*cos(the5)*sin(the3)*sin(the6) - a3*m6*the2_dot*y6*cos(the3)*cos(the4)*cos(the5)*sin(the2)*sin(the6) - a3*m6*the3_dot*y6*cos(the2)*cos(the4)*cos(the5)*sin(the3)*sin(the6) - a3*m6*the3_dot*y6*cos(the3)*cos(the4)*cos(the5)*sin(the2)*sin(the6) - a3*m6*the4_dot*y6*cos(the2)*cos(the3)*cos(the5)*sin(the4)*sin(the6) - a3*m6*the5_dot*y6*cos(the2)*cos(the3)*cos(the4)*sin(the5)*sin(the6) - a3*m6*the6_dot*y6*cos(the4)*cos(the5)*cos(the6)*sin(the2)*sin(the3) - d4*m6*the2_dot*x6*cos(the4)*cos(the5)*cos(the6)*sin(the2)*sin(the3) - d4*m6*the3_dot*x6*cos(the4)*cos(the5)*cos(the6)*sin(the2)*sin(the3) - d4*m6*the4_dot*x6*cos(the2)*cos(the5)*cos(the6)*sin(the3)*sin(the4) - d4*m6*the4_dot*x6*cos(the3)*cos(the5)*cos(the6)*sin(the2)*sin(the4) - d4*m6*the5_dot*x6*cos(the2)*cos(the4)*cos(the6)*sin(the3)*sin(the5) - d4*m6*the5_dot*x6*cos(the3)*cos(the4)*cos(the6)*sin(the2)*sin(the5) - d4*m6*the6_dot*x6*cos(the2)*cos(the4)*cos(the5)*sin(the3)*sin(the6) - d4*m6*the6_dot*x6*cos(the3)*cos(the4)*cos(the5)*sin(the2)*sin(the6) + m6*the2_dot*x6^2*cos(the6)*sin(the2)*sin(the3)*sin(the4)*sin(the5)*sin(the6) + m6*the3_dot*x6^2*cos(the6)*sin(the2)*sin(the3)*sin(the4)*sin(the5)*sin(the6) - m6*the2_dot*y6^2*cos(the6)*sin(the2)*sin(the3)*sin(the4)*sin(the5)*sin(the6) - m6*the3_dot*y6^2*cos(the6)*sin(the2)*sin(the3)*sin(the4)*sin(the5)*sin(the6) - m6*the2_dot*y6*z6*cos(the2)*cos(the3)*cos(the5)*cos(the6)*sin(the4) - m6*the3_dot*y6*z6*cos(the2)*cos(the3)*cos(the5)*cos(the6)*sin(the4) - m6*the4_dot*y6*z6*cos(the2)*cos(the4)*cos(the5)*cos(the6)*sin(the3) - m6*the4_dot*y6*z6*cos(the3)*cos(the4)*cos(the5)*cos(the6)*sin(the2) - 2*m6*the6_dot*y6*z6*cos(the2)*cos(the3)*cos(the5)*cos(the6)*sin(the5) - a3*m6*the4_dot*x6*cos(the5)*cos(the6)*sin(the2)*sin(the3)*sin(the4) - a3*m6*the5_dot*x6*cos(the4)*cos(the6)*sin(the2)*sin(the3)*sin(the5) - a3*m6*the6_dot*x6*cos(the4)*cos(the5)*sin(the2)*sin(the3)*sin(the6) + d4*m6*the2_dot*y6*cos(the4)*cos(the5)*sin(the2)*sin(the3)*sin(the6) + d4*m6*the3_dot*y6*cos(the4)*cos(the5)*sin(the2)*sin(the3)*sin(the6) + d4*m6*the4_dot*y6*cos(the2)*cos(the5)*sin(the3)*sin(the4)*sin(the6) + d4*m6*the4_dot*y6*cos(the3)*cos(the5)*sin(the2)*sin(the4)*sin(the6) + d4*m6*the5_dot*y6*cos(the2)*cos(the4)*sin(the3)*sin(the5)*sin(the6) + d4*m6*the5_dot*y6*cos(the3)*cos(the4)*sin(the2)*sin(the5)*sin(the6) - 4*m5*the5_dot*x5*y5*cos(the2)*cos(the4)*cos(the5)*sin(the3)*sin(the5) - 4*m5*the5_dot*x5*y5*cos(the3)*cos(the4)*cos(the5)*sin(the2)*sin(the5) + 2*m6*the6_dot*x6*y6*cos(the2)*cos(the4)*cos(the5)*sin(the3)*sin(the5) + 2*m6*the6_dot*x6*y6*cos(the3)*cos(the4)*cos(the5)*sin(the2)*sin(the5) + 2*m6*the5_dot*x6*y6*cos(the2)*cos(the4)*cos(the6)*sin(the3)*sin(the6) + 2*m6*the5_dot*x6*y6*cos(the3)*cos(the4)*cos(the6)*sin(the2)*sin(the6) - m6*the2_dot*x6*z6*cos(the2)*cos(the3)*cos(the5)*sin(the4)*sin(the6) - 2*m6*the2_dot*x6*z6*cos(the2)*cos(the5)*cos(the6)*sin(the3)*sin(the5) - 2*m6*the2_dot*x6*z6*cos(the3)*cos(the5)*cos(the6)*sin(the2)*sin(the5) - m6*the3_dot*x6*z6*cos(the2)*cos(the3)*cos(the5)*sin(the4)*sin(the6) - 2*m6*the3_dot*x6*z6*cos(the2)*cos(the5)*cos(the6)*sin(the3)*sin(the5) - 2*m6*the3_dot*x6*z6*cos(the3)*cos(the5)*cos(the6)*sin(the2)*sin(the5) - m6*the4_dot*x6*z6*cos(the2)*cos(the4)*cos(the5)*sin(the3)*sin(the6) - m6*the4_dot*x6*z6*cos(the3)*cos(the4)*cos(the5)*sin(the2)*sin(the6) - m6*the6_dot*x6*z6*cos(the2)*cos(the5)*cos(the6)*sin(the3)*sin(the4) - m6*the6_dot*x6*z6*cos(the3)*cos(the5)*cos(the6)*sin(the2)*sin(the4) - 2*m6*the6_dot*x6*z6*cos(the2)*cos(the3)*cos(the5)*sin(the5)*sin(the6) + a3*m6*the4_dot*y6*cos(the5)*sin(the2)*sin(the3)*sin(the4)*sin(the6) + a3*m6*the5_dot*y6*cos(the4)*sin(the2)*sin(the3)*sin(the5)*sin(the6) + m6*the2_dot*x6^2*cos(the2)*cos(the3)*cos(the4)*cos(the5)*cos(the6)^2*sin(the5) + m6*the3_dot*x6^2*cos(the2)*cos(the3)*cos(the4)*cos(the5)*cos(the6)^2*sin(the5) - m6*the2_dot*y6^2*cos(the2)*cos(the3)*cos(the4)*cos(the5)*cos(the6)^2*sin(the5) - m6*the3_dot*y6^2*cos(the2)*cos(the3)*cos(the4)*cos(the5)*cos(the6)^2*sin(the5) + m6*the2_dot*y6*z6*cos(the5)*cos(the6)*sin(the2)*sin(the3)*sin(the4) + 2*m6*the2_dot*y6*z6*cos(the2)*cos(the5)*sin(the3)*sin(the5)*sin(the6) + 2*m6*the2_dot*y6*z6*cos(the3)*cos(the5)*sin(the2)*sin(the5)*sin(the6) + m6*the3_dot*y6*z6*cos(the5)*cos(the6)*sin(the2)*sin(the3)*sin(the4) + 2*m6*the3_dot*y6*z6*cos(the2)*cos(the5)*sin(the3)*sin(the5)*sin(the6) + 2*m6*the3_dot*y6*z6*cos(the3)*cos(the5)*sin(the2)*sin(the5)*sin(the6) + m6*the5_dot*y6*z6*cos(the2)*cos(the6)*sin(the3)*sin(the4)*sin(the5) + m6*the5_dot*y6*z6*cos(the3)*cos(the6)*sin(the2)*sin(the4)*sin(the5) + m6*the6_dot*y6*z6*cos(the2)*cos(the5)*sin(the3)*sin(the4)*sin(the6) + m6*the6_dot*y6*z6*cos(the3)*cos(the5)*sin(the2)*sin(the4)*sin(the6) + 2*m6*the6_dot*y6*z6*cos(the5)*cos(the6)*sin(the2)*sin(the3)*sin(the5) + m6*the2_dot*x6*z6*cos(the5)*sin(the2)*sin(the3)*sin(the4)*sin(the6) + m6*the3_dot*x6*z6*cos(the5)*sin(the2)*sin(the3)*sin(the4)*sin(the6) + m6*the5_dot*x6*z6*cos(the2)*sin(the3)*sin(the4)*sin(the5)*sin(the6) + m6*the5_dot*x6*z6*cos(the3)*sin(the2)*sin(the4)*sin(the5)*sin(the6) + 2*m6*the6_dot*x6*z6*cos(the5)*sin(the2)*sin(the3)*sin(the5)*sin(the6) - m6*the2_dot*x6^2*cos(the4)*cos(the5)*cos(the6)^2*sin(the2)*sin(the3)*sin(the5) - m6*the3_dot*x6^2*cos(the4)*cos(the5)*cos(the6)^2*sin(the2)*sin(the3)*sin(the5) - m6*the4_dot*x6^2*cos(the2)*cos(the5)*cos(the6)^2*sin(the3)*sin(the4)*sin(the5) - m6*the4_dot*x6^2*cos(the3)*cos(the5)*cos(the6)^2*sin(the2)*sin(the4)*sin(the5) + m6*the2_dot*y6^2*cos(the4)*cos(the5)*cos(the6)^2*sin(the2)*sin(the3)*sin(the5) + m6*the3_dot*y6^2*cos(the4)*cos(the5)*cos(the6)^2*sin(the2)*sin(the3)*sin(the5) + m6*the4_dot*y6^2*cos(the2)*cos(the5)*cos(the6)^2*sin(the3)*sin(the4)*sin(the5) + m6*the4_dot*y6^2*cos(the3)*cos(the5)*cos(the6)^2*sin(the2)*sin(the4)*sin(the5) + 2*m6*the2_dot*x6*z6*cos(the2)*cos(the3)*cos(the4)*cos(the5)^2*cos(the6) + 2*m6*the3_dot*x6*z6*cos(the2)*cos(the3)*cos(the4)*cos(the5)^2*cos(the6) - 2*m6*the2_dot*y6*z6*cos(the2)*cos(the3)*cos(the4)*cos(the5)^2*sin(the6) - 2*m6*the3_dot*y6*z6*cos(the2)*cos(the3)*cos(the4)*cos(the5)^2*sin(the6) - 2*m6*the6_dot*y6*z6*cos(the2)*cos(the4)*cos(the5)^2*cos(the6)*sin(the3) - 2*m6*the6_dot*y6*z6*cos(the3)*cos(the4)*cos(the5)^2*cos(the6)*sin(the2) - 2*m6*the2_dot*x6*y6*cos(the2)*cos(the3)*cos(the6)^2*sin(the4)*sin(the5) - 2*m6*the3_dot*x6*y6*cos(the2)*cos(the3)*cos(the6)^2*sin(the4)*sin(the5) - 2*m6*the2_dot*x6*y6*cos(the2)*cos(the5)^2*cos(the6)*sin(the3)*sin(the6) - 2*m6*the2_dot*x6*y6*cos(the3)*cos(the5)^2*cos(the6)*sin(the2)*sin(the6) - 2*m6*the4_dot*x6*y6*cos(the2)*cos(the4)*cos(the6)^2*sin(the3)*sin(the5) - 2*m6*the4_dot*x6*y6*cos(the3)*cos(the4)*cos(the6)^2*sin(the2)*sin(the5) - 2*m6*the3_dot*x6*y6*cos(the2)*cos(the5)^2*cos(the6)*sin(the3)*sin(the6) - 2*m6*the3_dot*x6*y6*cos(the3)*cos(the5)^2*cos(the6)*sin(the2)*sin(the6) - 2*m6*the5_dot*x6*y6*cos(the2)*cos(the5)*cos(the6)^2*sin(the3)*sin(the4) - 2*m6*the5_dot*x6*y6*cos(the3)*cos(the5)*cos(the6)^2*sin(the2)*sin(the4) - 2*m6*the2_dot*x6*z6*cos(the4)*cos(the5)^2*cos(the6)*sin(the2)*sin(the3) - 2*m6*the3_dot*x6*z6*cos(the4)*cos(the5)^2*cos(the6)*sin(the2)*sin(the3) - 2*m6*the4_dot*x6*z6*cos(the2)*cos(the5)^2*cos(the6)*sin(the3)*sin(the4) - 2*m6*the4_dot*x6*z6*cos(the3)*cos(the5)^2*cos(the6)*sin(the2)*sin(the4) - 2*m6*the6_dot*x6*z6*cos(the2)*cos(the4)*cos(the5)^2*sin(the3)*sin(the6) - 2*m6*the6_dot*x6*z6*cos(the3)*cos(the4)*cos(the5)^2*sin(the2)*sin(the6) + 2*m6*the2_dot*y6*z6*cos(the4)*cos(the5)^2*sin(the2)*sin(the3)*sin(the6) + 2*m6*the3_dot*y6*z6*cos(the4)*cos(the5)^2*sin(the2)*sin(the3)*sin(the6) + 2*m6*the4_dot*y6*z6*cos(the2)*cos(the5)^2*sin(the3)*sin(the4)*sin(the6) + 2*m6*the4_dot*y6*z6*cos(the3)*cos(the5)^2*sin(the2)*sin(the4)*sin(the6) - 2*m6*the6_dot*x6^2*cos(the2)*cos(the4)*cos(the5)*cos(the6)*sin(the3)*sin(the5)*sin(the6) - 2*m6*the6_dot*x6^2*cos(the3)*cos(the4)*cos(the5)*cos(the6)*sin(the2)*sin(the5)*sin(the6) + 2*m6*the6_dot*y6^2*cos(the2)*cos(the4)*cos(the5)*cos(the6)*sin(the3)*sin(the5)*sin(the6) + 2*m6*the6_dot*y6^2*cos(the3)*cos(the4)*cos(the5)*cos(the6)*sin(the2)*sin(the5)*sin(the6) - 4*m6*the5_dot*x6*y6*cos(the2)*cos(the3)*cos(the5)*cos(the6)*sin(the5)*sin(the6) - 4*m6*the5_dot*x6*z6*cos(the2)*cos(the4)*cos(the5)*cos(the6)*sin(the3)*sin(the5) - 4*m6*the5_dot*x6*z6*cos(the3)*cos(the4)*cos(the5)*cos(the6)*sin(the2)*sin(the5) + 4*m6*the5_dot*y6*z6*cos(the2)*cos(the4)*cos(the5)*sin(the3)*sin(the5)*sin(the6) + 4*m6*the5_dot*y6*z6*cos(the3)*cos(the4)*cos(the5)*sin(the2)*sin(the5)*sin(the6) + 4*m6*the5_dot*x6*y6*cos(the5)*cos(the6)*sin(the2)*sin(the3)*sin(the5)*sin(the6) + 4*m6*the6_dot*x6*y6*cos(the2)*cos(the6)*sin(the3)*sin(the4)*sin(the5)*sin(the6) + 4*m6*the6_dot*x6*y6*cos(the3)*cos(the6)*sin(the2)*sin(the4)*sin(the5)*sin(the6) - 4*m6*the5_dot*x6*y6*cos(the2)*cos(the4)*cos(the5)^2*cos(the6)*sin(the3)*sin(the6) - 4*m6*the5_dot*x6*y6*cos(the3)*cos(the4)*cos(the5)^2*cos(the6)*sin(the2)*sin(the6) - 4*m6*the6_dot*x6*y6*cos(the2)*cos(the4)*cos(the5)*cos(the6)^2*sin(the3)*sin(the5) - 4*m6*the6_dot*x6*y6*cos(the3)*cos(the4)*cos(the5)*cos(the6)^2*sin(the2)*sin(the5) - 2*m6*the2_dot*x6*y6*cos(the2)*cos(the3)*cos(the4)*cos(the5)*cos(the6)*sin(the5)*sin(the6) - 2*m6*the3_dot*x6*y6*cos(the2)*cos(the3)*cos(the4)*cos(the5)*cos(the6)*sin(the5)*sin(the6) + 2*m6*the2_dot*x6*y6*cos(the4)*cos(the5)*cos(the6)*sin(the2)*sin(the3)*sin(the5)*sin(the6) + 2*m6*the3_dot*x6*y6*cos(the4)*cos(the5)*cos(the6)*sin(the2)*sin(the3)*sin(the5)*sin(the6) + 2*m6*the4_dot*x6*y6*cos(the2)*cos(the5)*cos(the6)*sin(the3)*sin(the4)*sin(the5)*sin(the6) + 2*m6*the4_dot*x6*y6*cos(the3)*cos(the5)*cos(the6)*sin(the2)*sin(the4)*sin(the5)*sin(the6),IPx6*the5_dot*cos(the2)*cos(the3)*cos(the5) + IPz5*the5_dot*cos(the2)*cos(the3)*cos(the5) - IPy5*the2_dot*cos(the2)*cos(the5)*sin(the3) - IPy5*the2_dot*cos(the3)*cos(the5)*sin(the2) - IPy5*the3_dot*cos(the2)*cos(the5)*sin(the3) - IPy5*the3_dot*cos(the3)*cos(the5)*sin(the2) - IPy5*the5_dot*cos(the2)*cos(the3)*sin(the5) - Ixx6*the2_dot*cos(the2)*cos(the3)*sin(the4) - Ixx6*the3_dot*cos(the2)*cos(the3)*sin(the4) - Ixx6*the4_dot*cos(the2)*cos(the4)*sin(the3) - Ixx6*the4_dot*cos(the3)*cos(the4)*sin(the2) - Ixx6*the6_dot*cos(the2)*cos(the3)*sin(the5) + Iyy6*the6_dot*cos(the2)*cos(the3)*sin(the5) - Izz5*the2_dot*cos(the2)*cos(the3)*sin(the4) - Izz5*the3_dot*cos(the2)*cos(the3)*sin(the4) - Izz5*the4_dot*cos(the2)*cos(the4)*sin(the3) - Izz5*the4_dot*cos(the3)*cos(the4)*sin(the2) - IPx6*the2_dot*cos(the2)*sin(the3)*sin(the5) - IPx6*the2_dot*cos(the3)*sin(the2)*sin(the5) - IPx6*the3_dot*cos(the2)*sin(the3)*sin(the5) - IPx6*the3_dot*cos(the3)*sin(the2)*sin(the5) - IPx6*the5_dot*cos(the5)*sin(the2)*sin(the3) - 2*IPx6*the6_dot*cos(the2)*sin(the3)*sin(the4) - 2*IPx6*the6_dot*cos(the3)*sin(the2)*sin(the4) - IPz5*the2_dot*cos(the2)*sin(the3)*sin(the5) - IPz5*the2_dot*cos(the3)*sin(the2)*sin(the5) - IPz5*the3_dot*cos(the2)*sin(the3)*sin(the5) - IPz5*the3_dot*cos(the3)*sin(the2)*sin(the5) - IPz5*the5_dot*cos(the5)*sin(the2)*sin(the3) + IPy5*the5_dot*sin(the2)*sin(the3)*sin(the5) + Ixx6*the2_dot*sin(the2)*sin(the3)*sin(the4) + Ixx6*the3_dot*sin(the2)*sin(the3)*sin(the4) + Ixx6*the6_dot*sin(the2)*sin(the3)*sin(the5) - Iyy6*the6_dot*sin(the2)*sin(the3)*sin(the5) + Izz5*the2_dot*sin(the2)*sin(the3)*sin(the4) + Izz5*the3_dot*sin(the2)*sin(the3)*sin(the4) - Ixx6*the2_dot*cos(the6)^2*sin(the2)*sin(the3)*sin(the4) - Ixx6*the3_dot*cos(the6)^2*sin(the2)*sin(the3)*sin(the4) - 2*Ixx6*the6_dot*cos(the6)^2*sin(the2)*sin(the3)*sin(the5) + Iyy6*the2_dot*cos(the6)^2*sin(the2)*sin(the3)*sin(the4) + Iyy6*the3_dot*cos(the6)^2*sin(the2)*sin(the3)*sin(the4) + 2*Iyy6*the6_dot*cos(the6)^2*sin(the2)*sin(the3)*sin(the5) + IPx6*the2_dot*cos(the2)*cos(the3)*cos(the4)*cos(the5) + IPx6*the3_dot*cos(the2)*cos(the3)*cos(the4)*cos(the5) + IPz5*the2_dot*cos(the2)*cos(the3)*cos(the4)*cos(the5) + IPz5*the3_dot*cos(the2)*cos(the3)*cos(the4)*cos(the5) - IPz6*the6_dot*cos(the2)*cos(the3)*cos(the5)*cos(the6) - IPy5*the2_dot*cos(the2)*cos(the3)*cos(the4)*sin(the5) - IPy5*the3_dot*cos(the2)*cos(the3)*cos(the4)*sin(the5) - IPy5*the5_dot*cos(the2)*cos(the4)*cos(the5)*sin(the3) - IPy5*the5_dot*cos(the3)*cos(the4)*cos(the5)*sin(the2) + IPy6*the2_dot*cos(the2)*cos(the5)*cos(the6)*sin(the3) + IPy6*the2_dot*cos(the3)*cos(the5)*cos(the6)*sin(the2) + IPy6*the3_dot*cos(the2)*cos(the5)*cos(the6)*sin(the3) + IPy6*the3_dot*cos(the3)*cos(the5)*cos(the6)*sin(the2) + IPy6*the5_dot*cos(the2)*cos(the3)*cos(the6)*sin(the5) + IPy6*the6_dot*cos(the2)*cos(the3)*cos(the5)*sin(the6) - Ixx6*the6_dot*cos(the2)*cos(the4)*cos(the5)*sin(the3) - Ixx6*the6_dot*cos(the3)*cos(the4)*cos(the5)*sin(the2) + Iyy6*the6_dot*cos(the2)*cos(the4)*cos(the5)*sin(the3) + Iyy6*the6_dot*cos(the3)*cos(the4)*cos(the5)*sin(the2) - IPx6*the2_dot*cos(the4)*cos(the5)*sin(the2)*sin(the3) - IPx6*the3_dot*cos(the4)*cos(the5)*sin(the2)*sin(the3) - IPx6*the4_dot*cos(the2)*cos(the5)*sin(the3)*sin(the4) - IPx6*the4_dot*cos(the3)*cos(the5)*sin(the2)*sin(the4) - IPx6*the5_dot*cos(the2)*cos(the4)*sin(the3)*sin(the5) - IPx6*the5_dot*cos(the3)*cos(the4)*sin(the2)*sin(the5) - IPz5*the2_dot*cos(the4)*cos(the5)*sin(the2)*sin(the3) - IPz5*the3_dot*cos(the4)*cos(the5)*sin(the2)*sin(the3) - IPz5*the4_dot*cos(the2)*cos(the5)*sin(the3)*sin(the4) - IPz5*the4_dot*cos(the3)*cos(the5)*sin(the2)*sin(the4) - IPz5*the5_dot*cos(the2)*cos(the4)*sin(the3)*sin(the5) - IPz5*the5_dot*cos(the3)*cos(the4)*sin(the2)*sin(the5) + IPz6*the2_dot*cos(the2)*cos(the5)*sin(the3)*sin(the6) + IPz6*the2_dot*cos(the3)*cos(the5)*sin(the2)*sin(the6) + IPz6*the3_dot*cos(the2)*cos(the5)*sin(the3)*sin(the6) + IPz6*the3_dot*cos(the3)*cos(the5)*sin(the2)*sin(the6) + IPz6*the5_dot*cos(the2)*cos(the3)*sin(the5)*sin(the6) + IPz6*the6_dot*cos(the5)*cos(the6)*sin(the2)*sin(the3) + IPy5*the2_dot*cos(the4)*sin(the2)*sin(the3)*sin(the5) + IPy5*the3_dot*cos(the4)*sin(the2)*sin(the3)*sin(the5) + IPy5*the4_dot*cos(the2)*sin(the3)*sin(the4)*sin(the5) + IPy5*the4_dot*cos(the3)*sin(the2)*sin(the4)*sin(the5) - IPy6*the5_dot*cos(the6)*sin(the2)*sin(the3)*sin(the5) - IPy6*the6_dot*cos(the5)*sin(the2)*sin(the3)*sin(the6) - m5*the2_dot*x5^2*cos(the2)*cos(the3)*sin(the4) - m5*the3_dot*x5^2*cos(the2)*cos(the3)*sin(the4) - m5*the4_dot*x5^2*cos(the2)*cos(the4)*sin(the3) - m5*the4_dot*x5^2*cos(the3)*cos(the4)*sin(the2) + m6*the6_dot*x6^2*cos(the2)*cos(the3)*sin(the5) - m5*the2_dot*y5^2*cos(the2)*cos(the3)*sin(the4) - m5*the3_dot*y5^2*cos(the2)*cos(the3)*sin(the4) - m5*the4_dot*y5^2*cos(the2)*cos(the4)*sin(the3) - m5*the4_dot*y5^2*cos(the3)*cos(the4)*sin(the2) - m6*the2_dot*y6^2*cos(the2)*cos(the3)*sin(the4) - m6*the3_dot*y6^2*cos(the2)*cos(the3)*sin(the4) - m6*the4_dot*y6^2*cos(the2)*cos(the4)*sin(the3) - m6*the4_dot*y6^2*cos(the3)*cos(the4)*sin(the2) - m6*the6_dot*y6^2*cos(the2)*cos(the3)*sin(the5) - m6*the2_dot*z6^2*cos(the2)*cos(the3)*sin(the4) - m6*the3_dot*z6^2*cos(the2)*cos(the3)*sin(the4) - m6*the4_dot*z6^2*cos(the2)*cos(the4)*sin(the3) - m6*the4_dot*z6^2*cos(the3)*cos(the4)*sin(the2) - IPz6*the5_dot*sin(the2)*sin(the3)*sin(the5)*sin(the6) + a1*m5*the4_dot*y5*cos(the4)*cos(the5) + a1*m6*the4_dot*z6*cos(the4)*cos(the5) + m5*the2_dot*x5^2*sin(the2)*sin(the3)*sin(the4) + m5*the3_dot*x5^2*sin(the2)*sin(the3)*sin(the4) - m6*the6_dot*x6^2*sin(the2)*sin(the3)*sin(the5) + m5*the2_dot*y5^2*sin(the2)*sin(the3)*sin(the4) + m5*the3_dot*y5^2*sin(the2)*sin(the3)*sin(the4) + m6*the2_dot*y6^2*sin(the2)*sin(the3)*sin(the4) + m6*the3_dot*y6^2*sin(the2)*sin(the3)*sin(the4) + m6*the6_dot*y6^2*sin(the2)*sin(the3)*sin(the5) + m6*the2_dot*z6^2*sin(the2)*sin(the3)*sin(the4) + m6*the3_dot*z6^2*sin(the2)*sin(the3)*sin(the4) + a1*m5*the4_dot*x5*cos(the4)*sin(the5) + a1*m5*the5_dot*x5*cos(the5)*sin(the4) - 2*IPx6*the5_dot*cos(the2)*cos(the3)*cos(the5)*cos(the6)^2 - a1*m5*the5_dot*y5*sin(the4)*sin(the5) - a1*m6*the5_dot*z6*sin(the4)*sin(the5) + Ixx6*the2_dot*cos(the2)*cos(the3)*cos(the6)^2*sin(the4) + Ixx6*the3_dot*cos(the2)*cos(the3)*cos(the6)^2*sin(the4) + Ixx6*the4_dot*cos(the2)*cos(the4)*cos(the6)^2*sin(the3) + Ixx6*the4_dot*cos(the3)*cos(the4)*cos(the6)^2*sin(the2) + 2*Ixx6*the6_dot*cos(the2)*cos(the3)*cos(the6)^2*sin(the5) - Iyy6*the2_dot*cos(the2)*cos(the3)*cos(the6)^2*sin(the4) - Iyy6*the3_dot*cos(the2)*cos(the3)*cos(the6)^2*sin(the4) - Iyy6*the4_dot*cos(the2)*cos(the4)*cos(the6)^2*sin(the3) - Iyy6*the4_dot*cos(the3)*cos(the4)*cos(the6)^2*sin(the2) - 2*Iyy6*the6_dot*cos(the2)*cos(the3)*cos(the6)^2*sin(the5) + 2*IPx6*the2_dot*cos(the2)*cos(the6)^2*sin(the3)*sin(the5) + 2*IPx6*the2_dot*cos(the3)*cos(the6)^2*sin(the2)*sin(the5) + 2*IPx6*the3_dot*cos(the2)*cos(the6)^2*sin(the3)*sin(the5) + 2*IPx6*the3_dot*cos(the3)*cos(the6)^2*sin(the2)*sin(the5) + 2*IPx6*the5_dot*cos(the5)*cos(the6)^2*sin(the2)*sin(the3) + 4*IPx6*the6_dot*cos(the2)*cos(the6)^2*sin(the3)*sin(the4) + 4*IPx6*the6_dot*cos(the3)*cos(the6)^2*sin(the2)*sin(the4) + m6*the2_dot*x6^2*cos(the6)^2*sin(the2)*sin(the3)*sin(the4) + m6*the3_dot*x6^2*cos(the6)^2*sin(the2)*sin(the3)*sin(the4) + 2*m6*the6_dot*x6^2*cos(the6)^2*sin(the2)*sin(the3)*sin(the5) - m6*the2_dot*y6^2*cos(the6)^2*sin(the2)*sin(the3)*sin(the4) - m6*the3_dot*y6^2*cos(the6)^2*sin(the2)*sin(the3)*sin(the4) - 2*m6*the6_dot*y6^2*cos(the6)^2*sin(the2)*sin(the3)*sin(the5) + IPy6*the2_dot*cos(the2)*cos(the3)*cos(the4)*cos(the6)*sin(the5) + IPy6*the3_dot*cos(the2)*cos(the3)*cos(the4)*cos(the6)*sin(the5) + IPy6*the5_dot*cos(the2)*cos(the4)*cos(the5)*cos(the6)*sin(the3) + IPy6*the5_dot*cos(the3)*cos(the4)*cos(the5)*cos(the6)*sin(the2) + Ixx6*the5_dot*cos(the2)*cos(the3)*cos(the5)*cos(the6)*sin(the6) - Iyy6*the5_dot*cos(the2)*cos(the3)*cos(the5)*cos(the6)*sin(the6) + 2*IPx6*the2_dot*cos(the2)*cos(the3)*cos(the6)*sin(the4)*sin(the6) + 2*IPx6*the3_dot*cos(the2)*cos(the3)*cos(the6)*sin(the4)*sin(the6) + 2*IPx6*the4_dot*cos(the2)*cos(the4)*cos(the6)*sin(the3)*sin(the6) + 2*IPx6*the4_dot*cos(the3)*cos(the4)*cos(the6)*sin(the2)*sin(the6) + 4*IPx6*the6_dot*cos(the2)*cos(the3)*cos(the6)*sin(the5)*sin(the6) + IPz6*the2_dot*cos(the2)*cos(the3)*cos(the4)*sin(the5)*sin(the6) + IPz6*the3_dot*cos(the2)*cos(the3)*cos(the4)*sin(the5)*sin(the6) + IPz6*the5_dot*cos(the2)*cos(the4)*cos(the5)*sin(the3)*sin(the6) + IPz6*the5_dot*cos(the3)*cos(the4)*cos(the5)*sin(the2)*sin(the6) + IPz6*the6_dot*cos(the2)*cos(the4)*cos(the6)*sin(the3)*sin(the5) + IPz6*the6_dot*cos(the3)*cos(the4)*cos(the6)*sin(the2)*sin(the5) - IPy6*the2_dot*cos(the4)*cos(the6)*sin(the2)*sin(the3)*sin(the5) - IPy6*the3_dot*cos(the4)*cos(the6)*sin(the2)*sin(the3)*sin(the5) - IPy6*the4_dot*cos(the2)*cos(the6)*sin(the3)*sin(the4)*sin(the5) - IPy6*the4_dot*cos(the3)*cos(the6)*sin(the2)*sin(the4)*sin(the5) - IPy6*the6_dot*cos(the2)*cos(the4)*sin(the3)*sin(the5)*sin(the6) - IPy6*the6_dot*cos(the3)*cos(the4)*sin(the2)*sin(the5)*sin(the6) - Ixx6*the2_dot*cos(the2)*cos(the6)*sin(the3)*sin(the5)*sin(the6) - Ixx6*the2_dot*cos(the3)*cos(the6)*sin(the2)*sin(the5)*sin(the6) - Ixx6*the3_dot*cos(the2)*cos(the6)*sin(the3)*sin(the5)*sin(the6) - Ixx6*the3_dot*cos(the3)*cos(the6)*sin(the2)*sin(the5)*sin(the6) - Ixx6*the5_dot*cos(the5)*cos(the6)*sin(the2)*sin(the3)*sin(the6) - 2*Ixx6*the6_dot*cos(the2)*cos(the6)*sin(the3)*sin(the4)*sin(the6) - 2*Ixx6*the6_dot*cos(the3)*cos(the6)*sin(the2)*sin(the4)*sin(the6) + Iyy6*the2_dot*cos(the2)*cos(the6)*sin(the3)*sin(the5)*sin(the6) + Iyy6*the2_dot*cos(the3)*cos(the6)*sin(the2)*sin(the5)*sin(the6) + Iyy6*the3_dot*cos(the2)*cos(the6)*sin(the3)*sin(the5)*sin(the6) + Iyy6*the3_dot*cos(the3)*cos(the6)*sin(the2)*sin(the5)*sin(the6) + Iyy6*the5_dot*cos(the5)*cos(the6)*sin(the2)*sin(the3)*sin(the6) + 2*Iyy6*the6_dot*cos(the2)*cos(the6)*sin(the3)*sin(the4)*sin(the6) + 2*Iyy6*the6_dot*cos(the3)*cos(the6)*sin(the2)*sin(the4)*sin(the6) + m6*the6_dot*x6^2*cos(the2)*cos(the4)*cos(the5)*sin(the3) + m6*the6_dot*x6^2*cos(the3)*cos(the4)*cos(the5)*sin(the2) - m6*the6_dot*y6^2*cos(the2)*cos(the4)*cos(the5)*sin(the3) - m6*the6_dot*y6^2*cos(the3)*cos(the4)*cos(the5)*sin(the2) - 2*IPx6*the2_dot*cos(the6)*sin(the2)*sin(the3)*sin(the4)*sin(the6) - 2*IPx6*the3_dot*cos(the6)*sin(the2)*sin(the3)*sin(the4)*sin(the6) - 4*IPx6*the6_dot*cos(the6)*sin(the2)*sin(the3)*sin(the5)*sin(the6) - IPz6*the2_dot*cos(the4)*sin(the2)*sin(the3)*sin(the5)*sin(the6) - IPz6*the3_dot*cos(the4)*sin(the2)*sin(the3)*sin(the5)*sin(the6) - IPz6*the4_dot*cos(the2)*sin(the3)*sin(the4)*sin(the5)*sin(the6) - IPz6*the4_dot*cos(the3)*sin(the2)*sin(the4)*sin(the5)*sin(the6) + a2*m5*the4_dot*y5*cos(the2)*cos(the4)*cos(the5) + a2*m6*the4_dot*z6*cos(the2)*cos(the4)*cos(the5) + a2*m5*the4_dot*x5*cos(the2)*cos(the4)*sin(the5) + a2*m5*the5_dot*x5*cos(the2)*cos(the5)*sin(the4) + a1*m6*the4_dot*x6*cos(the4)*cos(the6)*sin(the5) + a1*m6*the5_dot*x6*cos(the5)*cos(the6)*sin(the4) - 2*IPx6*the2_dot*cos(the2)*cos(the3)*cos(the4)*cos(the5)*cos(the6)^2 - 2*IPx6*the3_dot*cos(the2)*cos(the3)*cos(the4)*cos(the5)*cos(the6)^2 + m6*the5_dot*x6*y6*cos(the2)*cos(the3)*cos(the5) + m5*the5_dot*x5*z5*cos(the2)*cos(the3)*cos(the5) - a2*m5*the2_dot*y5*cos(the5)*sin(the2)*sin(the4) - a2*m5*the5_dot*y5*cos(the2)*sin(the4)*sin(the5) - a1*m6*the4_dot*y6*cos(the4)*sin(the5)*sin(the6) - a1*m6*the5_dot*y6*cos(the5)*sin(the4)*sin(the6) - a1*m6*the6_dot*y6*cos(the6)*sin(the4)*sin(the5) - a2*m6*the2_dot*z6*cos(the5)*sin(the2)*sin(the4) - a2*m6*the5_dot*z6*cos(the2)*sin(the4)*sin(the5) + 2*Ixx6*the6_dot*cos(the2)*cos(the4)*cos(the5)*cos(the6)^2*sin(the3) + 2*Ixx6*the6_dot*cos(the3)*cos(the4)*cos(the5)*cos(the6)^2*sin(the2) - 2*Iyy6*the6_dot*cos(the2)*cos(the4)*cos(the5)*cos(the6)^2*sin(the3) - 2*Iyy6*the6_dot*cos(the3)*cos(the4)*cos(the5)*cos(the6)^2*sin(the2) - m5*the2_dot*y5*z5*cos(the2)*cos(the5)*sin(the3) - m5*the2_dot*y5*z5*cos(the3)*cos(the5)*sin(the2) - m5*the3_dot*y5*z5*cos(the2)*cos(the5)*sin(the3) - m5*the3_dot*y5*z5*cos(the3)*cos(the5)*sin(the2) - m5*the5_dot*y5*z5*cos(the2)*cos(the3)*sin(the5) - a2*m5*the2_dot*x5*sin(the2)*sin(the4)*sin(the5) - a1*m6*the6_dot*x6*sin(the4)*sin(the5)*sin(the6) + 2*IPx6*the2_dot*cos(the4)*cos(the5)*cos(the6)^2*sin(the2)*sin(the3) + 2*IPx6*the3_dot*cos(the4)*cos(the5)*cos(the6)^2*sin(the2)*sin(the3) + 2*IPx6*the4_dot*cos(the2)*cos(the5)*cos(the6)^2*sin(the3)*sin(the4) + 2*IPx6*the4_dot*cos(the3)*cos(the5)*cos(the6)^2*sin(the2)*sin(the4) + 2*IPx6*the5_dot*cos(the2)*cos(the4)*cos(the6)^2*sin(the3)*sin(the5) + 2*IPx6*the5_dot*cos(the3)*cos(the4)*cos(the6)^2*sin(the2)*sin(the5) - m6*the2_dot*x6*y6*cos(the2)*sin(the3)*sin(the5) - m6*the2_dot*x6*y6*cos(the3)*sin(the2)*sin(the5) - m6*the3_dot*x6*y6*cos(the2)*sin(the3)*sin(the5) - m6*the3_dot*x6*y6*cos(the3)*sin(the2)*sin(the5) - m6*the5_dot*x6*y6*cos(the5)*sin(the2)*sin(the3) - 2*m6*the6_dot*x6*y6*cos(the2)*sin(the3)*sin(the4) - 2*m6*the6_dot*x6*y6*cos(the3)*sin(the2)*sin(the4) - m5*the2_dot*x5*z5*cos(the2)*sin(the3)*sin(the5) - m5*the2_dot*x5*z5*cos(the3)*sin(the2)*sin(the5) - m5*the3_dot*x5*z5*cos(the2)*sin(the3)*sin(the5) - m5*the3_dot*x5*z5*cos(the3)*sin(the2)*sin(the5) - m5*the5_dot*x5*z5*cos(the5)*sin(the2)*sin(the3) - m6*the2_dot*x6^2*cos(the2)*cos(the3)*cos(the6)^2*sin(the4) - m6*the3_dot*x6^2*cos(the2)*cos(the3)*cos(the6)^2*sin(the4) - m6*the4_dot*x6^2*cos(the2)*cos(the4)*cos(the6)^2*sin(the3) - m6*the4_dot*x6^2*cos(the3)*cos(the4)*cos(the6)^2*sin(the2) - 2*m6*the6_dot*x6^2*cos(the2)*cos(the3)*cos(the6)^2*sin(the5) + m6*the2_dot*y6^2*cos(the2)*cos(the3)*cos(the6)^2*sin(the4) + m6*the3_dot*y6^2*cos(the2)*cos(the3)*cos(the6)^2*sin(the4) + m6*the4_dot*y6^2*cos(the2)*cos(the4)*cos(the6)^2*sin(the3) + m6*the4_dot*y6^2*cos(the3)*cos(the4)*cos(the6)^2*sin(the2) + 2*m6*the6_dot*y6^2*cos(the2)*cos(the3)*cos(the6)^2*sin(the5) + m5*the5_dot*y5*z5*sin(the2)*sin(the3)*sin(the5) + 2*m6*the2_dot*x6*y6*cos(the2)*cos(the6)^2*sin(the3)*sin(the5) + 2*m6*the2_dot*x6*y6*cos(the3)*cos(the6)^2*sin(the2)*sin(the5) + 2*m6*the3_dot*x6*y6*cos(the2)*cos(the6)^2*sin(the3)*sin(the5) + 2*m6*the3_dot*x6*y6*cos(the3)*cos(the6)^2*sin(the2)*sin(the5) + 2*m6*the5_dot*x6*y6*cos(the5)*cos(the6)^2*sin(the2)*sin(the3) + 4*m6*the6_dot*x6*y6*cos(the2)*cos(the6)^2*sin(the3)*sin(the4) + 4*m6*the6_dot*x6*y6*cos(the3)*cos(the6)^2*sin(the2)*sin(the4) + Ixx6*the2_dot*cos(the2)*cos(the3)*cos(the4)*cos(the5)*cos(the6)*sin(the6) + Ixx6*the3_dot*cos(the2)*cos(the3)*cos(the4)*cos(the5)*cos(the6)*sin(the6) - Iyy6*the2_dot*cos(the2)*cos(the3)*cos(the4)*cos(the5)*cos(the6)*sin(the6) - Iyy6*the3_dot*cos(the2)*cos(the3)*cos(the4)*cos(the5)*cos(the6)*sin(the6) + 4*IPx6*the6_dot*cos(the2)*cos(the4)*cos(the5)*cos(the6)*sin(the3)*sin(the6) + 4*IPx6*the6_dot*cos(the3)*cos(the4)*cos(the5)*cos(the6)*sin(the2)*sin(the6) - Ixx6*the2_dot*cos(the4)*cos(the5)*cos(the6)*sin(the2)*sin(the3)*sin(the6) - Ixx6*the3_dot*cos(the4)*cos(the5)*cos(the6)*sin(the2)*sin(the3)*sin(the6) - Ixx6*the4_dot*cos(the2)*cos(the5)*cos(the6)*sin(the3)*sin(the4)*sin(the6) - Ixx6*the4_dot*cos(the3)*cos(the5)*cos(the6)*sin(the2)*sin(the4)*sin(the6) - Ixx6*the5_dot*cos(the2)*cos(the4)*cos(the6)*sin(the3)*sin(the5)*sin(the6) - Ixx6*the5_dot*cos(the3)*cos(the4)*cos(the6)*sin(the2)*sin(the5)*sin(the6) + Iyy6*the2_dot*cos(the4)*cos(the5)*cos(the6)*sin(the2)*sin(the3)*sin(the6) + Iyy6*the3_dot*cos(the4)*cos(the5)*cos(the6)*sin(the2)*sin(the3)*sin(the6) + Iyy6*the4_dot*cos(the2)*cos(the5)*cos(the6)*sin(the3)*sin(the4)*sin(the6) + Iyy6*the4_dot*cos(the3)*cos(the5)*cos(the6)*sin(the2)*sin(the4)*sin(the6) + Iyy6*the5_dot*cos(the2)*cos(the4)*cos(the6)*sin(the3)*sin(the5)*sin(the6) + Iyy6*the5_dot*cos(the3)*cos(the4)*cos(the6)*sin(the2)*sin(the5)*sin(the6) - m6*the5_dot*x6^2*cos(the2)*cos(the3)*cos(the5)*cos(the6)*sin(the6) + m6*the5_dot*y6^2*cos(the2)*cos(the3)*cos(the5)*cos(the6)*sin(the6) + a3*m5*the4_dot*y5*cos(the2)*cos(the3)*cos(the4)*cos(the5) + a3*m6*the4_dot*z6*cos(the2)*cos(the3)*cos(the4)*cos(the5) + m6*the2_dot*x6^2*cos(the2)*cos(the6)*sin(the3)*sin(the5)*sin(the6) + m6*the2_dot*x6^2*cos(the3)*cos(the6)*sin(the2)*sin(the5)*sin(the6) + m6*the3_dot*x6^2*cos(the2)*cos(the6)*sin(the3)*sin(the5)*sin(the6) + m6*the3_dot*x6^2*cos(the3)*cos(the6)*sin(the2)*sin(the5)*sin(the6) + m6*the5_dot*x6^2*cos(the5)*cos(the6)*sin(the2)*sin(the3)*sin(the6) + 2*m6*the6_dot*x6^2*cos(the2)*cos(the6)*sin(the3)*sin(the4)*sin(the6) + 2*m6*the6_dot*x6^2*cos(the3)*cos(the6)*sin(the2)*sin(the4)*sin(the6) - m6*the2_dot*y6^2*cos(the2)*cos(the6)*sin(the3)*sin(the5)*sin(the6) - m6*the2_dot*y6^2*cos(the3)*cos(the6)*sin(the2)*sin(the5)*sin(the6) - m6*the3_dot*y6^2*cos(the2)*cos(the6)*sin(the3)*sin(the5)*sin(the6) - m6*the3_dot*y6^2*cos(the3)*cos(the6)*sin(the2)*sin(the5)*sin(the6) - m6*the5_dot*y6^2*cos(the5)*cos(the6)*sin(the2)*sin(the3)*sin(the6) - 2*m6*the6_dot*y6^2*cos(the2)*cos(the6)*sin(the3)*sin(the4)*sin(the6) - 2*m6*the6_dot*y6^2*cos(the3)*cos(the6)*sin(the2)*sin(the4)*sin(the6) + a3*m5*the4_dot*x5*cos(the2)*cos(the3)*cos(the4)*sin(the5) + a3*m5*the5_dot*x5*cos(the2)*cos(the3)*cos(the5)*sin(the4) + a2*m6*the4_dot*x6*cos(the2)*cos(the4)*cos(the6)*sin(the5) + a2*m6*the5_dot*x6*cos(the2)*cos(the5)*cos(the6)*sin(the4) - d4*m5*the2_dot*y5*cos(the2)*cos(the3)*cos(the5)*sin(the4) - d4*m5*the3_dot*y5*cos(the2)*cos(the3)*cos(the5)*sin(the4) - d4*m5*the4_dot*y5*cos(the2)*cos(the4)*cos(the5)*sin(the3) - d4*m5*the4_dot*y5*cos(the3)*cos(the4)*cos(the5)*sin(the2) - d4*m6*the2_dot*z6*cos(the2)*cos(the3)*cos(the5)*sin(the4) - d4*m6*the3_dot*z6*cos(the2)*cos(the3)*cos(the5)*sin(the4) - d4*m6*the4_dot*z6*cos(the2)*cos(the4)*cos(the5)*sin(the3) - d4*m6*the4_dot*z6*cos(the3)*cos(the4)*cos(the5)*sin(the2) + m6*the2_dot*x6*y6*cos(the2)*cos(the3)*cos(the4)*cos(the5) + m6*the3_dot*x6*y6*cos(the2)*cos(the3)*cos(the4)*cos(the5) + m5*the2_dot*x5*z5*cos(the2)*cos(the3)*cos(the4)*cos(the5) + m5*the3_dot*x5*z5*cos(the2)*cos(the3)*cos(the4)*cos(the5) - m6*the6_dot*x6*z6*cos(the2)*cos(the3)*cos(the5)*cos(the6) - a3*m5*the2_dot*y5*cos(the2)*cos(the5)*sin(the3)*sin(the4) - a3*m5*the2_dot*y5*cos(the3)*cos(the5)*sin(the2)*sin(the4) - a3*m5*the3_dot*y5*cos(the2)*cos(the5)*sin(the3)*sin(the4) - a3*m5*the3_dot*y5*cos(the3)*cos(the5)*sin(the2)*sin(the4) - a3*m5*the4_dot*y5*cos(the4)*cos(the5)*sin(the2)*sin(the3) - a3*m5*the5_dot*y5*cos(the2)*cos(the3)*sin(the4)*sin(the5) - a2*m6*the4_dot*y6*cos(the2)*cos(the4)*sin(the5)*sin(the6) - a2*m6*the5_dot*y6*cos(the2)*cos(the5)*sin(the4)*sin(the6) - a2*m6*the6_dot*y6*cos(the2)*cos(the6)*sin(the4)*sin(the5) - a3*m6*the2_dot*z6*cos(the2)*cos(the5)*sin(the3)*sin(the4) - a3*m6*the2_dot*z6*cos(the3)*cos(the5)*sin(the2)*sin(the4) - a3*m6*the3_dot*z6*cos(the2)*cos(the5)*sin(the3)*sin(the4) - a3*m6*the3_dot*z6*cos(the3)*cos(the5)*sin(the2)*sin(the4) - a3*m6*the4_dot*z6*cos(the4)*cos(the5)*sin(the2)*sin(the3) - a3*m6*the5_dot*z6*cos(the2)*cos(the3)*sin(the4)*sin(the5) - d4*m5*the2_dot*x5*cos(the2)*cos(the3)*sin(the4)*sin(the5) - d4*m5*the3_dot*x5*cos(the2)*cos(the3)*sin(the4)*sin(the5) - d4*m5*the4_dot*x5*cos(the2)*cos(the4)*sin(the3)*sin(the5) - d4*m5*the4_dot*x5*cos(the3)*cos(the4)*sin(the2)*sin(the5) - d4*m5*the5_dot*x5*cos(the2)*cos(the5)*sin(the3)*sin(the4) - d4*m5*the5_dot*x5*cos(the3)*cos(the5)*sin(the2)*sin(the4) - m5*the2_dot*y5*z5*cos(the2)*cos(the3)*cos(the4)*sin(the5) - m5*the3_dot*y5*z5*cos(the2)*cos(the3)*cos(the4)*sin(the5) - m5*the5_dot*y5*z5*cos(the2)*cos(the4)*cos(the5)*sin(the3) - m5*the5_dot*y5*z5*cos(the3)*cos(the4)*cos(the5)*sin(the2) + m6*the2_dot*y6*z6*cos(the2)*cos(the5)*cos(the6)*sin(the3) + m6*the2_dot*y6*z6*cos(the3)*cos(the5)*cos(the6)*sin(the2) + m6*the3_dot*y6*z6*cos(the2)*cos(the5)*cos(the6)*sin(the3) + m6*the3_dot*y6*z6*cos(the3)*cos(the5)*cos(the6)*sin(the2) + m6*the5_dot*y6*z6*cos(the2)*cos(the3)*cos(the6)*sin(the5) + m6*the6_dot*y6*z6*cos(the2)*cos(the3)*cos(the5)*sin(the6) - a3*m5*the2_dot*x5*cos(the2)*sin(the3)*sin(the4)*sin(the5) - a3*m5*the2_dot*x5*cos(the3)*sin(the2)*sin(the4)*sin(the5) - a3*m5*the3_dot*x5*cos(the2)*sin(the3)*sin(the4)*sin(the5) - a3*m5*the3_dot*x5*cos(the3)*sin(the2)*sin(the4)*sin(the5) - a3*m5*the4_dot*x5*cos(the4)*sin(the2)*sin(the3)*sin(the5) - a3*m5*the5_dot*x5*cos(the5)*sin(the2)*sin(the3)*sin(the4) - a2*m6*the2_dot*x6*cos(the6)*sin(the2)*sin(the4)*sin(the5) - a2*m6*the6_dot*x6*cos(the2)*sin(the4)*sin(the5)*sin(the6) + d4*m5*the2_dot*y5*cos(the5)*sin(the2)*sin(the3)*sin(the4) + d4*m5*the3_dot*y5*cos(the5)*sin(the2)*sin(the3)*sin(the4) + d4*m5*the5_dot*y5*cos(the2)*sin(the3)*sin(the4)*sin(the5) + d4*m5*the5_dot*y5*cos(the3)*sin(the2)*sin(the4)*sin(the5) + d4*m6*the2_dot*z6*cos(the5)*sin(the2)*sin(the3)*sin(the4) + d4*m6*the3_dot*z6*cos(the5)*sin(the2)*sin(the3)*sin(the4) + d4*m6*the5_dot*z6*cos(the2)*sin(the3)*sin(the4)*sin(the5) + d4*m6*the5_dot*z6*cos(the3)*sin(the2)*sin(the4)*sin(the5) - m6*the2_dot*x6*y6*cos(the4)*cos(the5)*sin(the2)*sin(the3) - m6*the3_dot*x6*y6*cos(the4)*cos(the5)*sin(the2)*sin(the3) - m6*the4_dot*x6*y6*cos(the2)*cos(the5)*sin(the3)*sin(the4) - m6*the4_dot*x6*y6*cos(the3)*cos(the5)*sin(the2)*sin(the4) - m6*the5_dot*x6*y6*cos(the2)*cos(the4)*sin(the3)*sin(the5) - m6*the5_dot*x6*y6*cos(the3)*cos(the4)*sin(the2)*sin(the5) - m5*the2_dot*x5*z5*cos(the4)*cos(the5)*sin(the2)*sin(the3) - m5*the3_dot*x5*z5*cos(the4)*cos(the5)*sin(the2)*sin(the3) - m5*the4_dot*x5*z5*cos(the2)*cos(the5)*sin(the3)*sin(the4) - m5*the4_dot*x5*z5*cos(the3)*cos(the5)*sin(the2)*sin(the4) - m5*the5_dot*x5*z5*cos(the2)*cos(the4)*sin(the3)*sin(the5) - m5*the5_dot*x5*z5*cos(the3)*cos(the4)*sin(the2)*sin(the5) + m6*the2_dot*x6*z6*cos(the2)*cos(the5)*sin(the3)*sin(the6) + m6*the2_dot*x6*z6*cos(the3)*cos(the5)*sin(the2)*sin(the6) + m6*the3_dot*x6*z6*cos(the2)*cos(the5)*sin(the3)*sin(the6) + m6*the3_dot*x6*z6*cos(the3)*cos(the5)*sin(the2)*sin(the6) + m6*the5_dot*x6*z6*cos(the2)*cos(the3)*sin(the5)*sin(the6) + m6*the6_dot*x6*z6*cos(the5)*cos(the6)*sin(the2)*sin(the3) + a3*m5*the5_dot*y5*sin(the2)*sin(the3)*sin(the4)*sin(the5) + a2*m6*the2_dot*y6*sin(the2)*sin(the4)*sin(the5)*sin(the6) + a3*m6*the5_dot*z6*sin(the2)*sin(the3)*sin(the4)*sin(the5) + d4*m5*the2_dot*x5*sin(the2)*sin(the3)*sin(the4)*sin(the5) + d4*m5*the3_dot*x5*sin(the2)*sin(the3)*sin(the4)*sin(the5) - 2*m6*the6_dot*x6^2*cos(the2)*cos(the4)*cos(the5)*cos(the6)^2*sin(the3) - 2*m6*the6_dot*x6^2*cos(the3)*cos(the4)*cos(the5)*cos(the6)^2*sin(the2) + 2*m6*the6_dot*y6^2*cos(the2)*cos(the4)*cos(the5)*cos(the6)^2*sin(the3) + 2*m6*the6_dot*y6^2*cos(the3)*cos(the4)*cos(the5)*cos(the6)^2*sin(the2) + m5*the2_dot*y5*z5*cos(the4)*sin(the2)*sin(the3)*sin(the5) + m5*the3_dot*y5*z5*cos(the4)*sin(the2)*sin(the3)*sin(the5) + m5*the4_dot*y5*z5*cos(the2)*sin(the3)*sin(the4)*sin(the5) + m5*the4_dot*y5*z5*cos(the3)*sin(the2)*sin(the4)*sin(the5) - m6*the5_dot*y6*z6*cos(the6)*sin(the2)*sin(the3)*sin(the5) - m6*the6_dot*y6*z6*cos(the5)*sin(the2)*sin(the3)*sin(the6) - m6*the5_dot*x6*z6*sin(the2)*sin(the3)*sin(the5)*sin(the6) - 2*m6*the5_dot*x6*y6*cos(the2)*cos(the3)*cos(the5)*cos(the6)^2 - m6*the2_dot*x6^2*cos(the2)*cos(the3)*cos(the4)*cos(the5)*cos(the6)*sin(the6) - m6*the3_dot*x6^2*cos(the2)*cos(the3)*cos(the4)*cos(the5)*cos(the6)*sin(the6) + m6*the2_dot*y6^2*cos(the2)*cos(the3)*cos(the4)*cos(the5)*cos(the6)*sin(the6) + m6*the3_dot*y6^2*cos(the2)*cos(the3)*cos(the4)*cos(the5)*cos(the6)*sin(the6) + m6*the2_dot*x6^2*cos(the4)*cos(the5)*cos(the6)*sin(the2)*sin(the3)*sin(the6) + m6*the3_dot*x6^2*cos(the4)*cos(the5)*cos(the6)*sin(the2)*sin(the3)*sin(the6) + m6*the4_dot*x6^2*cos(the2)*cos(the5)*cos(the6)*sin(the3)*sin(the4)*sin(the6) + m6*the4_dot*x6^2*cos(the3)*cos(the5)*cos(the6)*sin(the2)*sin(the4)*sin(the6) + m6*the5_dot*x6^2*cos(the2)*cos(the4)*cos(the6)*sin(the3)*sin(the5)*sin(the6) + m6*the5_dot*x6^2*cos(the3)*cos(the4)*cos(the6)*sin(the2)*sin(the5)*sin(the6) - m6*the2_dot*y6^2*cos(the4)*cos(the5)*cos(the6)*sin(the2)*sin(the3)*sin(the6) - m6*the3_dot*y6^2*cos(the4)*cos(the5)*cos(the6)*sin(the2)*sin(the3)*sin(the6) - m6*the4_dot*y6^2*cos(the2)*cos(the5)*cos(the6)*sin(the3)*sin(the4)*sin(the6) - m6*the4_dot*y6^2*cos(the3)*cos(the5)*cos(the6)*sin(the2)*sin(the4)*sin(the6) - m6*the5_dot*y6^2*cos(the2)*cos(the4)*cos(the6)*sin(the3)*sin(the5)*sin(the6) - m6*the5_dot*y6^2*cos(the3)*cos(the4)*cos(the6)*sin(the2)*sin(the5)*sin(the6) + a3*m6*the4_dot*x6*cos(the2)*cos(the3)*cos(the4)*cos(the6)*sin(the5) + a3*m6*the5_dot*x6*cos(the2)*cos(the3)*cos(the5)*cos(the6)*sin(the4) - a3*m6*the4_dot*y6*cos(the2)*cos(the3)*cos(the4)*sin(the5)*sin(the6) - a3*m6*the5_dot*y6*cos(the2)*cos(the3)*cos(the5)*sin(the4)*sin(the6) - a3*m6*the6_dot*y6*cos(the2)*cos(the3)*cos(the6)*sin(the4)*sin(the5) - d4*m6*the2_dot*x6*cos(the2)*cos(the3)*cos(the6)*sin(the4)*sin(the5) - d4*m6*the3_dot*x6*cos(the2)*cos(the3)*cos(the6)*sin(the4)*sin(the5) - d4*m6*the4_dot*x6*cos(the2)*cos(the4)*cos(the6)*sin(the3)*sin(the5) - d4*m6*the4_dot*x6*cos(the3)*cos(the4)*cos(the6)*sin(the2)*sin(the5) - d4*m6*the5_dot*x6*cos(the2)*cos(the5)*cos(the6)*sin(the3)*sin(the4) - d4*m6*the5_dot*x6*cos(the3)*cos(the5)*cos(the6)*sin(the2)*sin(the4) + m6*the2_dot*y6*z6*cos(the2)*cos(the3)*cos(the4)*cos(the6)*sin(the5) + m6*the3_dot*y6*z6*cos(the2)*cos(the3)*cos(the4)*cos(the6)*sin(the5) + m6*the5_dot*y6*z6*cos(the2)*cos(the4)*cos(the5)*cos(the6)*sin(the3) + m6*the5_dot*y6*z6*cos(the3)*cos(the4)*cos(the5)*cos(the6)*sin(the2) - a3*m6*the2_dot*x6*cos(the2)*cos(the6)*sin(the3)*sin(the4)*sin(the5) - a3*m6*the2_dot*x6*cos(the3)*cos(the6)*sin(the2)*sin(the4)*sin(the5) - a3*m6*the3_dot*x6*cos(the2)*cos(the6)*sin(the3)*sin(the4)*sin(the5) - a3*m6*the3_dot*x6*cos(the3)*cos(the6)*sin(the2)*sin(the4)*sin(the5) - a3*m6*the4_dot*x6*cos(the4)*cos(the6)*sin(the2)*sin(the3)*sin(the5) - a3*m6*the5_dot*x6*cos(the5)*cos(the6)*sin(the2)*sin(the3)*sin(the4) - a3*m6*the6_dot*x6*cos(the2)*cos(the3)*sin(the4)*sin(the5)*sin(the6) + d4*m6*the2_dot*y6*cos(the2)*cos(the3)*sin(the4)*sin(the5)*sin(the6) + d4*m6*the3_dot*y6*cos(the2)*cos(the3)*sin(the4)*sin(the5)*sin(the6) + d4*m6*the4_dot*y6*cos(the2)*cos(the4)*sin(the3)*sin(the5)*sin(the6) + d4*m6*the4_dot*y6*cos(the3)*cos(the4)*sin(the2)*sin(the5)*sin(the6) + d4*m6*the5_dot*y6*cos(the2)*cos(the5)*sin(the3)*sin(the4)*sin(the6) + d4*m6*the5_dot*y6*cos(the3)*cos(the5)*sin(the2)*sin(the4)*sin(the6) + d4*m6*the6_dot*y6*cos(the2)*cos(the6)*sin(the3)*sin(the4)*sin(the5) + d4*m6*the6_dot*y6*cos(the3)*cos(the6)*sin(the2)*sin(the4)*sin(the5) + 2*m6*the2_dot*x6*y6*cos(the2)*cos(the3)*cos(the6)*sin(the4)*sin(the6) + 2*m6*the3_dot*x6*y6*cos(the2)*cos(the3)*cos(the6)*sin(the4)*sin(the6) + 2*m6*the4_dot*x6*y6*cos(the2)*cos(the4)*cos(the6)*sin(the3)*sin(the6) + 2*m6*the4_dot*x6*y6*cos(the3)*cos(the4)*cos(the6)*sin(the2)*sin(the6) + 4*m6*the6_dot*x6*y6*cos(the2)*cos(the3)*cos(the6)*sin(the5)*sin(the6) + m6*the2_dot*x6*z6*cos(the2)*cos(the3)*cos(the4)*sin(the5)*sin(the6) + m6*the3_dot*x6*z6*cos(the2)*cos(the3)*cos(the4)*sin(the5)*sin(the6) + m6*the5_dot*x6*z6*cos(the2)*cos(the4)*cos(the5)*sin(the3)*sin(the6) + m6*the5_dot*x6*z6*cos(the3)*cos(the4)*cos(the5)*sin(the2)*sin(the6) + m6*the6_dot*x6*z6*cos(the2)*cos(the4)*cos(the6)*sin(the3)*sin(the5) + m6*the6_dot*x6*z6*cos(the3)*cos(the4)*cos(the6)*sin(the2)*sin(the5) + a3*m6*the2_dot*y6*cos(the2)*sin(the3)*sin(the4)*sin(the5)*sin(the6) + a3*m6*the2_dot*y6*cos(the3)*sin(the2)*sin(the4)*sin(the5)*sin(the6) + a3*m6*the3_dot*y6*cos(the2)*sin(the3)*sin(the4)*sin(the5)*sin(the6) + a3*m6*the3_dot*y6*cos(the3)*sin(the2)*sin(the4)*sin(the5)*sin(the6) + a3*m6*the4_dot*y6*cos(the4)*sin(the2)*sin(the3)*sin(the5)*sin(the6) + a3*m6*the5_dot*y6*cos(the5)*sin(the2)*sin(the3)*sin(the4)*sin(the6) + a3*m6*the6_dot*y6*cos(the6)*sin(the2)*sin(the3)*sin(the4)*sin(the5) + d4*m6*the2_dot*x6*cos(the6)*sin(the2)*sin(the3)*sin(the4)*sin(the5) + d4*m6*the3_dot*x6*cos(the6)*sin(the2)*sin(the3)*sin(the4)*sin(the5) + d4*m6*the6_dot*x6*cos(the2)*sin(the3)*sin(the4)*sin(the5)*sin(the6) + d4*m6*the6_dot*x6*cos(the3)*sin(the2)*sin(the4)*sin(the5)*sin(the6) - m6*the2_dot*y6*z6*cos(the4)*cos(the6)*sin(the2)*sin(the3)*sin(the5) - m6*the3_dot*y6*z6*cos(the4)*cos(the6)*sin(the2)*sin(the3)*sin(the5) - m6*the4_dot*y6*z6*cos(the2)*cos(the6)*sin(the3)*sin(the4)*sin(the5) - m6*the4_dot*y6*z6*cos(the3)*cos(the6)*sin(the2)*sin(the4)*sin(the5) - m6*the6_dot*y6*z6*cos(the2)*cos(the4)*sin(the3)*sin(the5)*sin(the6) - m6*the6_dot*y6*z6*cos(the3)*cos(the4)*sin(the2)*sin(the5)*sin(the6) + a3*m6*the6_dot*x6*sin(the2)*sin(the3)*sin(the4)*sin(the5)*sin(the6) - d4*m6*the2_dot*y6*sin(the2)*sin(the3)*sin(the4)*sin(the5)*sin(the6) - d4*m6*the3_dot*y6*sin(the2)*sin(the3)*sin(the4)*sin(the5)*sin(the6) - 2*m6*the2_dot*x6*y6*cos(the6)*sin(the2)*sin(the3)*sin(the4)*sin(the6) - 2*m6*the3_dot*x6*y6*cos(the6)*sin(the2)*sin(the3)*sin(the4)*sin(the6) - 4*m6*the6_dot*x6*y6*cos(the6)*sin(the2)*sin(the3)*sin(the5)*sin(the6) - m6*the2_dot*x6*z6*cos(the4)*sin(the2)*sin(the3)*sin(the5)*sin(the6) - m6*the3_dot*x6*z6*cos(the4)*sin(the2)*sin(the3)*sin(the5)*sin(the6) - m6*the4_dot*x6*z6*cos(the2)*sin(the3)*sin(the4)*sin(the5)*sin(the6) - m6*the4_dot*x6*z6*cos(the3)*sin(the2)*sin(the4)*sin(the5)*sin(the6) - 2*m6*the2_dot*x6*y6*cos(the2)*cos(the3)*cos(the4)*cos(the5)*cos(the6)^2 - 2*m6*the3_dot*x6*y6*cos(the2)*cos(the3)*cos(the4)*cos(the5)*cos(the6)^2 + 2*m6*the2_dot*x6*y6*cos(the4)*cos(the5)*cos(the6)^2*sin(the2)*sin(the3) + 2*m6*the3_dot*x6*y6*cos(the4)*cos(the5)*cos(the6)^2*sin(the2)*sin(the3) + 2*m6*the4_dot*x6*y6*cos(the2)*cos(the5)*cos(the6)^2*sin(the3)*sin(the4) + 2*m6*the4_dot*x6*y6*cos(the3)*cos(the5)*cos(the6)^2*sin(the2)*sin(the4) + 2*m6*the5_dot*x6*y6*cos(the2)*cos(the4)*cos(the6)^2*sin(the3)*sin(the5) + 2*m6*the5_dot*x6*y6*cos(the3)*cos(the4)*cos(the6)^2*sin(the2)*sin(the5) + 4*m6*the6_dot*x6*y6*cos(the2)*cos(the4)*cos(the5)*cos(the6)*sin(the3)*sin(the6) + 4*m6*the6_dot*x6*y6*cos(the3)*cos(the4)*cos(the5)*cos(the6)*sin(the2)*sin(the6),Izz6*the2_dot*cos(the2)*cos(the5)*sin(the3) + Izz6*the2_dot*cos(the3)*cos(the5)*sin(the2) + Izz6*the3_dot*cos(the2)*cos(the5)*sin(the3) + Izz6*the3_dot*cos(the3)*cos(the5)*sin(the2) + Izz6*the5_dot*cos(the2)*cos(the3)*sin(the5) - Izz6*the5_dot*sin(the2)*sin(the3)*sin(the5) + IPz6*the5_dot*cos(the2)*cos(the3)*cos(the5)*cos(the6) - IPy6*the2_dot*cos(the2)*cos(the3)*cos(the6)*sin(the4) - IPy6*the3_dot*cos(the2)*cos(the3)*cos(the6)*sin(the4) - IPy6*the4_dot*cos(the2)*cos(the4)*cos(the6)*sin(the3) - IPy6*the4_dot*cos(the3)*cos(the4)*cos(the6)*sin(the2) - IPy6*the5_dot*cos(the2)*cos(the3)*cos(the5)*sin(the6) - IPy6*the6_dot*cos(the2)*cos(the3)*cos(the6)*sin(the5) + Izz6*the2_dot*cos(the2)*cos(the3)*cos(the4)*sin(the5) + Izz6*the3_dot*cos(the2)*cos(the3)*cos(the4)*sin(the5) + Izz6*the5_dot*cos(the2)*cos(the4)*cos(the5)*sin(the3) + Izz6*the5_dot*cos(the3)*cos(the4)*cos(the5)*sin(the2) - IPz6*the2_dot*cos(the2)*cos(the3)*sin(the4)*sin(the6) - IPz6*the2_dot*cos(the2)*cos(the6)*sin(the3)*sin(the5) - IPz6*the2_dot*cos(the3)*cos(the6)*sin(the2)*sin(the5) - IPz6*the3_dot*cos(the2)*cos(the3)*sin(the4)*sin(the6) - IPz6*the3_dot*cos(the2)*cos(the6)*sin(the3)*sin(the5) - IPz6*the3_dot*cos(the3)*cos(the6)*sin(the2)*sin(the5) - IPz6*the4_dot*cos(the2)*cos(the4)*sin(the3)*sin(the6) - IPz6*the4_dot*cos(the3)*cos(the4)*sin(the2)*sin(the6) - IPz6*the5_dot*cos(the5)*cos(the6)*sin(the2)*sin(the3) - IPz6*the6_dot*cos(the2)*cos(the6)*sin(the3)*sin(the4) - IPz6*the6_dot*cos(the3)*cos(the6)*sin(the2)*sin(the4) - IPz6*the6_dot*cos(the2)*cos(the3)*sin(the5)*sin(the6) + IPy6*the2_dot*cos(the6)*sin(the2)*sin(the3)*sin(the4) + IPy6*the2_dot*cos(the2)*sin(the3)*sin(the5)*sin(the6) + IPy6*the2_dot*cos(the3)*sin(the2)*sin(the5)*sin(the6) + IPy6*the3_dot*cos(the6)*sin(the2)*sin(the3)*sin(the4) + IPy6*the3_dot*cos(the2)*sin(the3)*sin(the5)*sin(the6) + IPy6*the3_dot*cos(the3)*sin(the2)*sin(the5)*sin(the6) + IPy6*the5_dot*cos(the5)*sin(the2)*sin(the3)*sin(the6) + IPy6*the6_dot*cos(the2)*sin(the3)*sin(the4)*sin(the6) + IPy6*the6_dot*cos(the3)*sin(the2)*sin(the4)*sin(the6) + IPy6*the6_dot*cos(the6)*sin(the2)*sin(the3)*sin(the5) - Izz6*the2_dot*cos(the4)*sin(the2)*sin(the3)*sin(the5) - Izz6*the3_dot*cos(the4)*sin(the2)*sin(the3)*sin(the5) - Izz6*the4_dot*cos(the2)*sin(the3)*sin(the4)*sin(the5) - Izz6*the4_dot*cos(the3)*sin(the2)*sin(the4)*sin(the5) + m6*the2_dot*x6^2*cos(the2)*cos(the5)*sin(the3) + m6*the2_dot*x6^2*cos(the3)*cos(the5)*sin(the2) + m6*the3_dot*x6^2*cos(the2)*cos(the5)*sin(the3) + m6*the3_dot*x6^2*cos(the3)*cos(the5)*sin(the2) + m6*the5_dot*x6^2*cos(the2)*cos(the3)*sin(the5) + m6*the2_dot*y6^2*cos(the2)*cos(the5)*sin(the3) + m6*the2_dot*y6^2*cos(the3)*cos(the5)*sin(the2) + m6*the3_dot*y6^2*cos(the2)*cos(the5)*sin(the3) + m6*the3_dot*y6^2*cos(the3)*cos(the5)*sin(the2) + m6*the5_dot*y6^2*cos(the2)*cos(the3)*sin(the5) + IPz6*the2_dot*sin(the2)*sin(the3)*sin(the4)*sin(the6) + IPz6*the3_dot*sin(the2)*sin(the3)*sin(the4)*sin(the6) + IPz6*the6_dot*sin(the2)*sin(the3)*sin(the5)*sin(the6) + a1*m6*the6_dot*y6*cos(the4)*cos(the6) - m6*the5_dot*x6^2*sin(the2)*sin(the3)*sin(the5) - m6*the5_dot*y6^2*sin(the2)*sin(the3)*sin(the5) + a1*m6*the4_dot*x6*cos(the6)*sin(the4) + a1*m6*the6_dot*x6*cos(the4)*sin(the6) - a1*m6*the4_dot*y6*sin(the4)*sin(the6) + IPz6*the2_dot*cos(the2)*cos(the3)*cos(the4)*cos(the5)*cos(the6) + IPz6*the3_dot*cos(the2)*cos(the3)*cos(the4)*cos(the5)*cos(the6) - IPy6*the2_dot*cos(the2)*cos(the3)*cos(the4)*cos(the5)*sin(the6) - IPy6*the3_dot*cos(the2)*cos(the3)*cos(the4)*cos(the5)*sin(the6) - IPy6*the6_dot*cos(the2)*cos(the4)*cos(the5)*cos(the6)*sin(the3) - IPy6*the6_dot*cos(the3)*cos(the4)*cos(the5)*cos(the6)*sin(the2) - IPz6*the2_dot*cos(the4)*cos(the5)*cos(the6)*sin(the2)*sin(the3) - IPz6*the3_dot*cos(the4)*cos(the5)*cos(the6)*sin(the2)*sin(the3) - IPz6*the4_dot*cos(the2)*cos(the5)*cos(the6)*sin(the3)*sin(the4) - IPz6*the4_dot*cos(the3)*cos(the5)*cos(the6)*sin(the2)*sin(the4) - IPz6*the5_dot*cos(the2)*cos(the4)*cos(the6)*sin(the3)*sin(the5) - IPz6*the5_dot*cos(the3)*cos(the4)*cos(the6)*sin(the2)*sin(the5) - IPz6*the6_dot*cos(the2)*cos(the4)*cos(the5)*sin(the3)*sin(the6) - IPz6*the6_dot*cos(the3)*cos(the4)*cos(the5)*sin(the2)*sin(the6) + IPy6*the2_dot*cos(the4)*cos(the5)*sin(the2)*sin(the3)*sin(the6) + IPy6*the3_dot*cos(the4)*cos(the5)*sin(the2)*sin(the3)*sin(the6) + IPy6*the4_dot*cos(the2)*cos(the5)*sin(the3)*sin(the4)*sin(the6) + IPy6*the4_dot*cos(the3)*cos(the5)*sin(the2)*sin(the4)*sin(the6) + IPy6*the5_dot*cos(the2)*cos(the4)*sin(the3)*sin(the5)*sin(the6) + IPy6*the5_dot*cos(the3)*cos(the4)*sin(the2)*sin(the5)*sin(the6) + m6*the2_dot*x6^2*cos(the2)*cos(the3)*cos(the4)*sin(the5) + m6*the3_dot*x6^2*cos(the2)*cos(the3)*cos(the4)*sin(the5) + m6*the5_dot*x6^2*cos(the2)*cos(the4)*cos(the5)*sin(the3) + m6*the5_dot*x6^2*cos(the3)*cos(the4)*cos(the5)*sin(the2) + m6*the2_dot*y6^2*cos(the2)*cos(the3)*cos(the4)*sin(the5) + m6*the3_dot*y6^2*cos(the2)*cos(the3)*cos(the4)*sin(the5) + m6*the5_dot*y6^2*cos(the2)*cos(the4)*cos(the5)*sin(the3) + m6*the5_dot*y6^2*cos(the3)*cos(the4)*cos(the5)*sin(the2) + a1*m6*the4_dot*y6*cos(the4)*cos(the5)*cos(the6) + a2*m6*the6_dot*y6*cos(the2)*cos(the4)*cos(the6) - m6*the2_dot*x6^2*cos(the4)*sin(the2)*sin(the3)*sin(the5) - m6*the3_dot*x6^2*cos(the4)*sin(the2)*sin(the3)*sin(the5) - m6*the4_dot*x6^2*cos(the2)*sin(the3)*sin(the4)*sin(the5) - m6*the4_dot*x6^2*cos(the3)*sin(the2)*sin(the4)*sin(the5) - m6*the2_dot*y6^2*cos(the4)*sin(the2)*sin(the3)*sin(the5) - m6*the3_dot*y6^2*cos(the4)*sin(the2)*sin(the3)*sin(the5) - m6*the4_dot*y6^2*cos(the2)*sin(the3)*sin(the4)*sin(the5) - m6*the4_dot*y6^2*cos(the3)*sin(the2)*sin(the4)*sin(the5) + a2*m6*the2_dot*x6*cos(the4)*cos(the6)*sin(the2) + a2*m6*the4_dot*x6*cos(the2)*cos(the6)*sin(the4) + a1*m6*the4_dot*x6*cos(the4)*cos(the5)*sin(the6) + a2*m6*the6_dot*x6*cos(the2)*cos(the4)*sin(the6) + a1*m6*the6_dot*x6*cos(the5)*cos(the6)*sin(the4) - a2*m6*the2_dot*y6*cos(the4)*sin(the2)*sin(the6) - a2*m6*the4_dot*y6*cos(the2)*sin(the4)*sin(the6) - a1*m6*the5_dot*y6*cos(the6)*sin(the4)*sin(the5) - a1*m6*the6_dot*y6*cos(the5)*sin(the4)*sin(the6) - a1*m6*the5_dot*x6*sin(the4)*sin(the5)*sin(the6) + a2*m6*the4_dot*y6*cos(the2)*cos(the4)*cos(the5)*cos(the6) + a3*m6*the6_dot*y6*cos(the2)*cos(the3)*cos(the4)*cos(the6) + d4*m6*the2_dot*x6*cos(the2)*cos(the3)*cos(the4)*cos(the6) + d4*m6*the3_dot*x6*cos(the2)*cos(the3)*cos(the4)*cos(the6) + a3*m6*the2_dot*x6*cos(the2)*cos(the4)*cos(the6)*sin(the3) + a3*m6*the2_dot*x6*cos(the3)*cos(the4)*cos(the6)*sin(the2) + a3*m6*the3_dot*x6*cos(the2)*cos(the4)*cos(the6)*sin(the3) + a3*m6*the3_dot*x6*cos(the3)*cos(the4)*cos(the6)*sin(the2) + a3*m6*the4_dot*x6*cos(the2)*cos(the3)*cos(the6)*sin(the4) + a2*m6*the4_dot*x6*cos(the2)*cos(the4)*cos(the5)*sin(the6) + a3*m6*the6_dot*x6*cos(the2)*cos(the3)*cos(the4)*sin(the6) + a2*m6*the6_dot*x6*cos(the2)*cos(the5)*cos(the6)*sin(the4) - d4*m6*the2_dot*y6*cos(the2)*cos(the3)*cos(the4)*sin(the6) - d4*m6*the3_dot*y6*cos(the2)*cos(the3)*cos(the4)*sin(the6) - d4*m6*the6_dot*y6*cos(the2)*cos(the4)*cos(the6)*sin(the3) - d4*m6*the6_dot*y6*cos(the3)*cos(the4)*cos(the6)*sin(the2) + m6*the5_dot*x6*z6*cos(the2)*cos(the3)*cos(the5)*cos(the6) - a3*m6*the2_dot*y6*cos(the2)*cos(the4)*sin(the3)*sin(the6) - a3*m6*the2_dot*y6*cos(the3)*cos(the4)*sin(the2)*sin(the6) - a2*m6*the2_dot*y6*cos(the5)*cos(the6)*sin(the2)*sin(the4) - a3*m6*the3_dot*y6*cos(the2)*cos(the4)*sin(the3)*sin(the6) - a3*m6*the3_dot*y6*cos(the3)*cos(the4)*sin(the2)*sin(the6) - a3*m6*the4_dot*y6*cos(the2)*cos(the3)*sin(the4)*sin(the6) - a2*m6*the5_dot*y6*cos(the2)*cos(the6)*sin(the4)*sin(the5) - a3*m6*the6_dot*y6*cos(the4)*cos(the6)*sin(the2)*sin(the3) - a2*m6*the6_dot*y6*cos(the2)*cos(the5)*sin(the4)*sin(the6) - d4*m6*the2_dot*x6*cos(the4)*cos(the6)*sin(the2)*sin(the3) - d4*m6*the3_dot*x6*cos(the4)*cos(the6)*sin(the2)*sin(the3) - d4*m6*the4_dot*x6*cos(the2)*cos(the6)*sin(the3)*sin(the4) - d4*m6*the4_dot*x6*cos(the3)*cos(the6)*sin(the2)*sin(the4) - d4*m6*the6_dot*x6*cos(the2)*cos(the4)*sin(the3)*sin(the6) - d4*m6*the6_dot*x6*cos(the3)*cos(the4)*sin(the2)*sin(the6) - m6*the2_dot*y6*z6*cos(the2)*cos(the3)*cos(the6)*sin(the4) - m6*the3_dot*y6*z6*cos(the2)*cos(the3)*cos(the6)*sin(the4) - m6*the4_dot*y6*z6*cos(the2)*cos(the4)*cos(the6)*sin(the3) - m6*the4_dot*y6*z6*cos(the3)*cos(the4)*cos(the6)*sin(the2) - m6*the5_dot*y6*z6*cos(the2)*cos(the3)*cos(the5)*sin(the6) - m6*the6_dot*y6*z6*cos(the2)*cos(the3)*cos(the6)*sin(the5) - a2*m6*the2_dot*x6*cos(the5)*sin(the2)*sin(the4)*sin(the6) - a3*m6*the4_dot*x6*cos(the6)*sin(the2)*sin(the3)*sin(the4) - a2*m6*the5_dot*x6*cos(the2)*sin(the4)*sin(the5)*sin(the6) - a3*m6*the6_dot*x6*cos(the4)*sin(the2)*sin(the3)*sin(the6) + d4*m6*the2_dot*y6*cos(the4)*sin(the2)*sin(the3)*sin(the6) + d4*m6*the3_dot*y6*cos(the4)*sin(the2)*sin(the3)*sin(the6) + d4*m6*the4_dot*y6*cos(the2)*sin(the3)*sin(the4)*sin(the6) + d4*m6*the4_dot*y6*cos(the3)*sin(the2)*sin(the4)*sin(the6) - m6*the2_dot*x6*z6*cos(the2)*cos(the3)*sin(the4)*sin(the6) - m6*the2_dot*x6*z6*cos(the2)*cos(the6)*sin(the3)*sin(the5) - m6*the2_dot*x6*z6*cos(the3)*cos(the6)*sin(the2)*sin(the5) - m6*the3_dot*x6*z6*cos(the2)*cos(the3)*sin(the4)*sin(the6) - m6*the3_dot*x6*z6*cos(the2)*cos(the6)*sin(the3)*sin(the5) - m6*the3_dot*x6*z6*cos(the3)*cos(the6)*sin(the2)*sin(the5) - m6*the4_dot*x6*z6*cos(the2)*cos(the4)*sin(the3)*sin(the6) - m6*the4_dot*x6*z6*cos(the3)*cos(the4)*sin(the2)*sin(the6) - m6*the5_dot*x6*z6*cos(the5)*cos(the6)*sin(the2)*sin(the3) - m6*the6_dot*x6*z6*cos(the2)*cos(the6)*sin(the3)*sin(the4) - m6*the6_dot*x6*z6*cos(the3)*cos(the6)*sin(the2)*sin(the4) - m6*the6_dot*x6*z6*cos(the2)*cos(the3)*sin(the5)*sin(the6) + a3*m6*the4_dot*y6*sin(the2)*sin(the3)*sin(the4)*sin(the6) + m6*the2_dot*y6*z6*cos(the6)*sin(the2)*sin(the3)*sin(the4) + m6*the2_dot*y6*z6*cos(the2)*sin(the3)*sin(the5)*sin(the6) + m6*the2_dot*y6*z6*cos(the3)*sin(the2)*sin(the5)*sin(the6) + m6*the3_dot*y6*z6*cos(the6)*sin(the2)*sin(the3)*sin(the4) + m6*the3_dot*y6*z6*cos(the2)*sin(the3)*sin(the5)*sin(the6) + m6*the3_dot*y6*z6*cos(the3)*sin(the2)*sin(the5)*sin(the6) + m6*the5_dot*y6*z6*cos(the5)*sin(the2)*sin(the3)*sin(the6) + m6*the6_dot*y6*z6*cos(the2)*sin(the3)*sin(the4)*sin(the6) + m6*the6_dot*y6*z6*cos(the3)*sin(the2)*sin(the4)*sin(the6) + m6*the6_dot*y6*z6*cos(the6)*sin(the2)*sin(the3)*sin(the5) + m6*the2_dot*x6*z6*sin(the2)*sin(the3)*sin(the4)*sin(the6) + m6*the3_dot*x6*z6*sin(the2)*sin(the3)*sin(the4)*sin(the6) + m6*the6_dot*x6*z6*sin(the2)*sin(the3)*sin(the5)*sin(the6) + a3*m6*the4_dot*y6*cos(the2)*cos(the3)*cos(the4)*cos(the5)*cos(the6) + a3*m6*the4_dot*x6*cos(the2)*cos(the3)*cos(the4)*cos(the5)*sin(the6) + a3*m6*the6_dot*x6*cos(the2)*cos(the3)*cos(the5)*cos(the6)*sin(the4) - d4*m6*the2_dot*y6*cos(the2)*cos(the3)*cos(the5)*cos(the6)*sin(the4) - d4*m6*the3_dot*y6*cos(the2)*cos(the3)*cos(the5)*cos(the6)*sin(the4) - d4*m6*the4_dot*y6*cos(the2)*cos(the4)*cos(the5)*cos(the6)*sin(the3) - d4*m6*the4_dot*y6*cos(the3)*cos(the4)*cos(the5)*cos(the6)*sin(the2) + m6*the2_dot*x6*z6*cos(the2)*cos(the3)*cos(the4)*cos(the5)*cos(the6) + m6*the3_dot*x6*z6*cos(the2)*cos(the3)*cos(the4)*cos(the5)*cos(the6) - a3*m6*the2_dot*y6*cos(the2)*cos(the5)*cos(the6)*sin(the3)*sin(the4) - a3*m6*the2_dot*y6*cos(the3)*cos(the5)*cos(the6)*sin(the2)*sin(the4) - a3*m6*the3_dot*y6*cos(the2)*cos(the5)*cos(the6)*sin(the3)*sin(the4) - a3*m6*the3_dot*y6*cos(the3)*cos(the5)*cos(the6)*sin(the2)*sin(the4) - a3*m6*the4_dot*y6*cos(the4)*cos(the5)*cos(the6)*sin(the2)*sin(the3) - a3*m6*the5_dot*y6*cos(the2)*cos(the3)*cos(the6)*sin(the4)*sin(the5) - a3*m6*the6_dot*y6*cos(the2)*cos(the3)*cos(the5)*sin(the4)*sin(the6) - d4*m6*the2_dot*x6*cos(the2)*cos(the3)*cos(the5)*sin(the4)*sin(the6) - d4*m6*the3_dot*x6*cos(the2)*cos(the3)*cos(the5)*sin(the4)*sin(the6) - d4*m6*the4_dot*x6*cos(the2)*cos(the4)*cos(the5)*sin(the3)*sin(the6) - d4*m6*the4_dot*x6*cos(the3)*cos(the4)*cos(the5)*sin(the2)*sin(the6) - d4*m6*the6_dot*x6*cos(the2)*cos(the5)*cos(the6)*sin(the3)*sin(the4) - d4*m6*the6_dot*x6*cos(the3)*cos(the5)*cos(the6)*sin(the2)*sin(the4) - m6*the2_dot*y6*z6*cos(the2)*cos(the3)*cos(the4)*cos(the5)*sin(the6) - m6*the3_dot*y6*z6*cos(the2)*cos(the3)*cos(the4)*cos(the5)*sin(the6) - m6*the6_dot*y6*z6*cos(the2)*cos(the4)*cos(the5)*cos(the6)*sin(the3) - m6*the6_dot*y6*z6*cos(the3)*cos(the4)*cos(the5)*cos(the6)*sin(the2) - a3*m6*the2_dot*x6*cos(the2)*cos(the5)*sin(the3)*sin(the4)*sin(the6) - a3*m6*the2_dot*x6*cos(the3)*cos(the5)*sin(the2)*sin(the4)*sin(the6) - a3*m6*the3_dot*x6*cos(the2)*cos(the5)*sin(the3)*sin(the4)*sin(the6) - a3*m6*the3_dot*x6*cos(the3)*cos(the5)*sin(the2)*sin(the4)*sin(the6) - a3*m6*the4_dot*x6*cos(the4)*cos(the5)*sin(the2)*sin(the3)*sin(the6) - a3*m6*the5_dot*x6*cos(the2)*cos(the3)*sin(the4)*sin(the5)*sin(the6) - a3*m6*the6_dot*x6*cos(the5)*cos(the6)*sin(the2)*sin(the3)*sin(the4) + d4*m6*the2_dot*y6*cos(the5)*cos(the6)*sin(the2)*sin(the3)*sin(the4) + d4*m6*the3_dot*y6*cos(the5)*cos(the6)*sin(the2)*sin(the3)*sin(the4) + d4*m6*the5_dot*y6*cos(the2)*cos(the6)*sin(the3)*sin(the4)*sin(the5) + d4*m6*the5_dot*y6*cos(the3)*cos(the6)*sin(the2)*sin(the4)*sin(the5) + d4*m6*the6_dot*y6*cos(the2)*cos(the5)*sin(the3)*sin(the4)*sin(the6) + d4*m6*the6_dot*y6*cos(the3)*cos(the5)*sin(the2)*sin(the4)*sin(the6) - m6*the2_dot*x6*z6*cos(the4)*cos(the5)*cos(the6)*sin(the2)*sin(the3) - m6*the3_dot*x6*z6*cos(the4)*cos(the5)*cos(the6)*sin(the2)*sin(the3) - m6*the4_dot*x6*z6*cos(the2)*cos(the5)*cos(the6)*sin(the3)*sin(the4) - m6*the4_dot*x6*z6*cos(the3)*cos(the5)*cos(the6)*sin(the2)*sin(the4) - m6*the5_dot*x6*z6*cos(the2)*cos(the4)*cos(the6)*sin(the3)*sin(the5) - m6*the5_dot*x6*z6*cos(the3)*cos(the4)*cos(the6)*sin(the2)*sin(the5) - m6*the6_dot*x6*z6*cos(the2)*cos(the4)*cos(the5)*sin(the3)*sin(the6) - m6*the6_dot*x6*z6*cos(the3)*cos(the4)*cos(the5)*sin(the2)*sin(the6) + a3*m6*the5_dot*y6*cos(the6)*sin(the2)*sin(the3)*sin(the4)*sin(the5) + a3*m6*the6_dot*y6*cos(the5)*sin(the2)*sin(the3)*sin(the4)*sin(the6) + d4*m6*the2_dot*x6*cos(the5)*sin(the2)*sin(the3)*sin(the4)*sin(the6) + d4*m6*the3_dot*x6*cos(the5)*sin(the2)*sin(the3)*sin(the4)*sin(the6) + d4*m6*the5_dot*x6*cos(the2)*sin(the3)*sin(the4)*sin(the5)*sin(the6) + d4*m6*the5_dot*x6*cos(the3)*sin(the2)*sin(the4)*sin(the5)*sin(the6) + m6*the2_dot*y6*z6*cos(the4)*cos(the5)*sin(the2)*sin(the3)*sin(the6) + m6*the3_dot*y6*z6*cos(the4)*cos(the5)*sin(the2)*sin(the3)*sin(the6) + m6*the4_dot*y6*z6*cos(the2)*cos(the5)*sin(the3)*sin(the4)*sin(the6) + m6*the4_dot*y6*z6*cos(the3)*cos(the5)*sin(the2)*sin(the4)*sin(the6) + m6*the5_dot*y6*z6*cos(the2)*cos(the4)*sin(the3)*sin(the5)*sin(the6) + m6*the5_dot*y6*z6*cos(the3)*cos(the4)*sin(the2)*sin(the5)*sin(the6) + a3*m6*the5_dot*x6*sin(the2)*sin(the3)*sin(the4)*sin(the5)*sin(the6);
